simulink model "FullFMS_2026_02_25_V0_4_8"  (R2026a)
settings: Solver=FixedStepAuto  StopTime=inf  FixedStep=0.01  MaxStep=0.01  RelTol=1e-2
PreLoadFcn:
  | load("BUS_CONFIG.mat")
libraries: opcualib x8
(part 3 of 5)

== stateflow chart FullFMS_2026_02_25_V0_4_8/Chart ==
  state Variable_Declaration
    state VarDeclaration_20
      entry:
      %Actuators
      Actuators_20.F_22_Led_On;
      Actuators_20.F_22_Led_Off;
      Actuators_20.F_22_Conveyor;
      Actuators_20.F_24_Release_FB;
      Actuators_20.F_25_Release_FB;
      Actuators_20.F_26_Release_FB;
      Actuators_20.F_27_Release_FB;
      Actuators_20.F_28_Release_FB;
      Actuators_20.F_29_Release_FB;
      %Control
      Control_20.C_24_CartDel;
      Control_20.C_24_CRoute_Out;
      Control_20.C_24_Request;
      Control_20.C_24_CRoute_In;
      Control_20.C_25_CartDel;
      Control_20.C_25_CRoute_Out;
      Control_20.C_25_Request;
      Control_20.C_25_CRoute_In;
      Control_20.C_26_CartDel;
      Control_20.C_26_CRoute_Out;
      Control_20.C_26_Request;
      Control_20.C_26_CRoute_In;
      Control_20.C_27_CartDel;
      Control_20.C_27_CRoute_Out;
      Control_20.C_27_Request;
      Control_20.C_27_CRoute_In;
      Control_20.C_28_CartDel;
      Control_20.C_28_CRoute_Out;
      Control_20.C_28_Request;
      Control_20.C_28_CRoute_In;
      Control_20.C_29_CartDel;
      Control_20.C_29_CRoute_Out;
      Control_20.C_29_Request;
      Control_20.C_29_CRoute_In;
      %Sensors
      Sensors_20.O_20_On;
      Sensors_20.O_20_Off;
      Sensors_20.O_20_Controler_On;
      Sensors_20.O_24_Cart_Stat;
      Sensors_20.O_24_Cart_Next;
      Sensors_20.O_24_Optic;
      Sensors_20.O_24_Count;
      Sensors_20.O_24_Pist_Bck;
      Sensors_20.O_25_Cart_Stat;
      Sensors_20.O_25_Cart_Next;
      Sensors_20.O_25_Optic;
      Sensors_20.O_25_Count;
      Sensors_20.O_25_Pist_Bck;
      Sensors_20.O_26_Cart_Stat;
      Sensors_20.O_26_Cart_Next;
      Sensors_20.O_26_Optic;
      Sensors_20.O_26_Count;
      Sensors_20.O_26_Pist_Bck;
      Sensors_20.O_27_Cart_Stat;
      Sensors_20.O_27_Cart_Next;
      Sensors_20.O_27_Optic;
      Sensors_20.O_27_Count;
      Sensors_20.O_27_Pist_Bck;
      Sensors_20.O_28_Cart_Stat;
      Sensors_20.O_28_Cart_Next;
      Sensors_20.O_28_Optic;
      Sensors_20.O_28_Count;
      Sensors_20.O_28_Pist_Bck;
      Sensors_20.O_29_Cart_Stat;
      Sensors_20.O_29_Cart_Next;
      Sensors_20.O_29_Optic;
      Sensors_20.O_29_Count;
      Sensors_20.O_29_Pist_Bck;
    state VarDeclaration_30
      entry:
      %Actuators
      Actuators_30.F_33_Led_Start;
      Actuators_30.F_33_Led_Reset;
      Actuators_30.F_33_Led_Extra1;
      Actuators_30.F_33_Led_Extra2;
      Actuators_30.F_33_Spring_Cyl;
      Actuators_30.F_33_Cover_Cyl;
      %AS-i
      AS_i_30.A_34_Request;
      AS_i_30.A_34_No_Cart;
      AS_i_30.A_34_Cart_Full;
      AS_i_30.A_34_CRoute_Out;
      AS_i_30.A_32_RoboCartID;
      AS_i_30.A_34_Cart_Stat;
      AS_i_30.A_34_Cart_Next;
      AS_i_30.A_34_Optic;
      AS_i_30.A_34_Count;
      AS_i_30.A_34_Pist_Bck;
      AS_i_30.A_34_Release_FB;
      AS_i_30.A_34_CRoute_In;
      %Control
      Control_30.C_30_Robot1;
      Control_30.C_30_Robot2;
      Control_30.C_35_Part_Del;
      %Sensors
      Sensors_30.O_31_Start;
      Sensors_30.O_31_Stop;
      Sensors_30.O_31_Reset;
      Sensors_30.O_31_Part_in_Claw;
      Sensors_30.O_31_Orientation;
      Sensors_30.O_32_Sp_Cyl_Bck;
      Sensors_30.O_32_Sp_Cyl_Fwd;
      Sensors_30.O_32_Co_Cyl_Bck;
      Sensors_30.O_32_Co_Cyl_Fwd;
      Sensors_30.O_32_Sp_PickUp;
      Sensors_30.O_32_Co_PickUp;
      Sensors_30.O_32_CoMag_Empty;
    state VarDeclaration_40
      entry:
      %Actuators
      Actuators_40.F_43_Led_Start;
      Actuators_40.F_43_Led_Reset;
      Actuators_40.F_43_Led_Extra1;
      Actuators_40.F_43_Led_Extra2;
      Actuators_40.F_43_Panel_O4;
      Actuators_40.F_43_Panel_O5;
      Actuators_40.F_43_Panel_O6;
      Actuators_40.F_43_Panel_O7;
      %AS-i
      AS_i_40.A_44_Request;
      AS_i_40.A_44_No_Cart;
      AS_i_40.A_44_Cart_Full;
      AS_i_40.A_44_CRoute_Out;
      AS_i_40.A_43_StorCartID;
      AS_i_40.A_44_Cart_Stat;
      AS_i_40.A_44_Cart_Next;
      AS_i_40.A_44_Optic;
      AS_i_40.A_44_Count;
      AS_i_40.A_44_Pist_Bck;
      AS_i_40.A_44_Release_FB;
      AS_i_40.A_44_CRoute_In;
      %Control
      Control_40.C_45_Initialization;
      Control_40.C_42_Profibus;
      Control_40.C_45_Start;
      Control_40.C_45_StorePart;
      Control_40.C_45_RetrievePart;
      %Sensors
      Sensors_40.O_41_Start;
      Sensors_40.O_41_Stop;
      Sensors_40.O_41_Key_Pos;
      Sensors_40.O_41_Reset;
      Sensors_40.O_41_Panel_I4;
      Sensors_40.O_41_Panel_I5;
      Sensors_40.O_41_Panel_I6;
      Sensors_40.O_41_Panel_I7;
    state VarDeclaration_50
      entry:
      %Actuators
      Actuators_50.F_52_Claw_2_Del;
      Actuators_50.F_52_Claw_2_Cart;
      Actuators_50.F_52_Claw_Down;
      Actuators_50.F_52_Close_Claw;
      Actuators_50.F_53_Led_Start;
      Actuators_50.F_53_Led_Reset;
      Actuators_50.F_53_Led_Extra1;
      Actuators_50.F_53_Led_Extra2;
      Actuators_50.F_53_Panel_O4;
      Actuators_50.F_53_Panel_O5;
      Actuators_50.F_53_Panel_O6;
      Actuators_50.F_53_Panel_O7;
      %AS-i
      AS_i_50.A_54_Request;
      AS_i_50.A_54_No_Cart;
      AS_i_50.A_54_Cart_Full;
      AS_i_50.A_54_CRoute_Out;
      AS_i_50.A_53_SortCartID;
      AS_i_50.A_54_Cart_Stat;
      AS_i_50.A_54_Cart_Next;
      AS_i_50.A_54_Optic;
      AS_i_50.A_54_Count;
      AS_i_50.A_54_Pist_Bck;
      AS_i_50.A_54_Release_FB;
      AS_i_50.A_54_CRoute_In;
      %Control
      Control_50.C_55_Initialization;
      Control_50.C_55_PD_Sort;
      Control_50.C_52_Profibus;
      Control_50.C_55_Start;
      Control_50.C_55_Cart2Del;
      %Sensors
      Sensors_50.O_50_Part_Reserve;
      Sensors_50.O_50_Claw_Cart;
      Sensors_50.O_50_Claw_Del;
      Sensors_50.O_50_Claw_Reserve;
      Sensors_50.O_50_Claw_Low;
      Sensors_50.O_50_Claw_High;
      Sensors_50.O_50_Part_in_Claw;
      Sensors_50.O_51_Start;
      Sensors_50.O_51_Stop;
      Sensors_50.O_51_Key_Pos;
      Sensors_50.O_51_Reset;
      Sensors_50.O_51_Panel_I4;
      Sensors_50.O_51_Panel_I5;
      Sensors_50.O_51_Panel_I6;
      Sensors_50.O_51_Panel_I7;
    state VarDeclaration_60
      entry:
      %Actuators
      Actuators_60.F_62_Conveyor;
      Actuators_60.F_62_P1;
      Actuators_60.F_62_P2;
      Actuators_60.F_62_Identify;
      Actuators_60.F_63_Led_Start;
      Actuators_60.F_63_Led_Reset;
      Actuators_60.F_63_Led_Extra1;
      Actuators_60.F_63_Led_Extra2;
      Actuators_60.F_63_Panel_O4;
      Actuators_60.F_63_Panel_O5;
      Actuators_60.F_63_Panel_O6;
      Actuators_60.F_63_Panel_O7;
      %Control
      Control_60.C_65_Initialization;
      Control_60.C_65_ID_1;
      Control_60.C_65_ID_2;
      Control_60.C_65_Part_Sorted;
      Control_60.C_62_Profibus;
      Control_60.C_65_RBS_Output;
      Control_60.C_65_RSB_Output;
      Control_60.C_65_BRS_Output;
      Control_60.C_65_BSR_Output;
      Control_60.C_65_SRB_Output;
      Control_60.C_65_SBR_Output;
      %Sensors
      Sensors_60.O_60_SPart;
      Sensors_60.O_60_SInd;
      Sensors_60.O_60_SPhoto;
      Sensors_60.O_60_Part_Pass;
      Sensors_60.O_60_SL1_Bck;
      Sensors_60.O_60_SL1_Fwd;
      Sensors_60.O_60_SL2_Bck;
      Sensors_60.O_60_SL2_Fwd;
      Sensors_60.O_61_Start;
      Sensors_60.O_61_Stop;
      Sensors_60.O_61_Key_Pos;
      Sensors_60.O_61_Reset;
      Sensors_60.O_61_Panel_I4;
      Sensors_60.O_61_Panel_I5;
      Sensors_60.O_61_Panel_I6;
      Sensors_60.O_61_Panel_I7;
    state VarDeclaration_70
      entry:
      %Actuators
      Actuators_70.F_72_Elev_Down;
      Actuators_70.F_72_Elev_Up;
      Actuators_70.F_72_Eject_Part;
      Actuators_70.F_72_Air_On;
      Actuators_70.F_73_Led_Start;
      Actuators_70.F_73_Led_Reset;
      Actuators_70.F_73_Led_Extra1;
      Actuators_70.F_73_Led_Extra2;
      Actuators_70.F_73_Panel_O4;
      Actuators_70.F_73_Panel_O5;
      Actuators_70.F_73_Panel_O6;
      Actuators_70.F_73_Panel_O7;
      %AS-i
      AS_i_70.A_74_Request;
      AS_i_70.A_74_No_Cart;
      AS_i_70.A_74_Cart_Full;
      AS_i_70.A_74_CRoute_Out;
      AS_i_70.A_74_CRoute_In80;
      AS_i_70.A_73_TestCartID;
      AS_i_70.A_74_Cart_Stat;
      AS_i_70.A_74_Cart_Next;
      AS_i_70.A_74_Optic;
      AS_i_70.A_74_Count;
      AS_i_70.A_74_Pist_Bck;
      AS_i_70.A_74_Release_FB;
      AS_i_70.A_74_CRoute_In;
      %Control
      Control_70.C_75_Initialization;
      Control_70.C_75_ID_Delivery1;
      Control_70.C_75_ID_Delivery2;
      Control_70.C_75_Part_Del;
      Control_70.C_75_RQ_Part_Del;
      Control_70.C_75_RQ_Wrong;
      Control_70.C_75_Identified80;
      Control_70.C_75_Requested80;
      Control_70.C_72_Profibus;
      Control_70.C_75_RQ_Delivery1;
      Control_70.C_75_RQ_Delivery2;
      Control_70.C_75_Identified;
      Control_70.C_75_Requested;
      %Sensors
      Sensors_70.O_70_SInductive;
      Sensors_70.O_70_SPart;
      Sensors_70.O_70_SStation;
      Sensors_70.O_70_SPart_Height;
      Sensors_70.O_70_Elev_High;
      Sensors_70.O_70_Elev_Low;
      Sensors_70.O_70_Pist_Bck;
      Sensors_70.O_71_Start;
      Sensors_70.O_71_Stop;
      Sensors_70.O_71_Key_Pos;
      Sensors_70.O_71_Reset;
      Sensors_70.O_71_Panel_I4;
      Sensors_70.O_71_Panel_I5;
      Sensors_70.O_71_Panel_I6;
      Sensors_70.O_71_Panel_I7;
    state VarDeclaration_80
      entry:
      %Actuators
      Actuators_80.F_82_Pist_Adv;
      Actuators_80.F_82_Suction_On;
      Actuators_80.F_82_Suction_Off;
      Actuators_80.F_82_Arm_2_Del;
      Actuators_80.F_82_Arm_2_Mag;
      Actuators_80.F_83_Led_Start;
      Actuators_80.F_83_Led_Reset;
      Actuators_80.F_83_Led_Extra1;
      Actuators_80.F_83_Led_Extra2;
      Actuators_80.F_83_Panel_O4;
      Actuators_80.F_83_Panel_O5;
      Actuators_80.F_83_Panel_O6;
      Actuators_80.F_83_Panel_O7;
      %Control
      Control_80.C_85_Initialization;
      Control_80.C_85_Part_Del;
      Control_80.C_85_Part_Mag;
      Control_80.C_86_Mag_Parts;
      Control_80.C_87_RQ_MParts;
      Control_80.C_82_Profibus;
      Control_80.C_83_RQ_Parts;
      Control_80.C_85_Start;
      Control_80.C_85_Single;
      Control_80.C_85_Continuous;
      Control_80.C_85_Counted;
      %Sensors
      Sensors_80.O_80_Mag_Full;
      Sensors_80.O_80_Pist_Bck;
      Sensors_80.O_80_Pist_Fwd;
      Sensors_80.O_80_Part_Stuck;
      Sensors_80.O_80_Arm_Mag;
      Sensors_80.O_80_Arm_Del;
      Sensors_80.O_80_Mag_Empty;
      Sensors_80.O_81_Start;
      Sensors_80.O_81_Stop;,
      Sensors_80.O_81_Key_Pos;
      Sensors_80.O_81_Reset;
      Sensors_80.O_81_Panel_I4;
      Sensors_80.O_81_Panel_I5;
      Sensors_80.O_81_Panel_I6;
      Sensors_80.O_81_Panel_I7;
    state VarDeclaration_90
      entry:
      %Actuators
      Actuators_90.F_92_Claw_2_Cart;
      Actuators_90.F_92_Claw_2_Del;
      Actuators_90.F_92_Claw_Down;
      Actuators_90.F_92_Close_Claw;
      Actuators_90.F_93_Led_Start;
      Actuators_90.F_93_Led_Reset;
      Actuators_90.F_93_Led_Extra1;
      Actuators_90.F_93_Led_Extra2;
      Actuators_90.F_93_Panel_O4;
      Actuators_90.F_93_Panel_O5;
      Actuators_90.F_93_Panel_O6;
      Actuators_90.F_93_Panel_O7;
      %AS-i
      AS_i_90.A_94_Request;
      AS_i_90.A_94_No_Cart;
      AS_i_90.A_94_Cart_Full;
      AS_i_90.A_94_CRoute_Out;
      AS_i_90.A_93_ProcCartID;
      AS_i_90.A_94_Cart_Stat;
      AS_i_90.A_94_Cart_Next;
      AS_i_90.A_94_Optic;
      AS_i_90.A_94_Count;
      AS_i_90.A_94_Pist_Bck;
      AS_i_90.A_94_Release_FB;
      AS_i_90.A_94_CRoute_In;
      %Control
      Control_90.C_95_Initialization;
      Control_90.C_95_PD_Proc;
      Control_90.C_95_PD_Cart;
      Control_90.C_92_Profibus;
      Control_90.C_95_Start;
      Control_90.C_95_Cart2Del;
      Control_90.C_95_Del2Cart;
      %Sensors
      Sensors_90.O_90_Part_Reserve;
      Sensors_90.O_90_Claw_Del;
      Sensors_90.O_90_Claw_Cart;
      Sensors_90.O_90_Claw_Reserve;
      Sensors_90.O_90_Claw_Low;
      Sensors_90.O_90_Claw_High;
      Sensors_90.O_90_Part_in_Claw;
      Sensors_90.O_91_Start;
      Sensors_90.O_91_Stop;
      Sensors_90.O_91_Key_Pos;
      Sensors_90.O_91_Reset;
      Sensors_90.O_91_Panel_I4;
      Sensors_90.O_91_Panel_I5;
      Sensors_90.O_91_Panel_I6;
      Sensors_90.O_91_Panel_I7;
    state VarDeclaration_100
      entry:
      %Actuators
      Actuators_100.F_102_Drill_On;
      Actuators_100.F_102_RT_On;
      Actuators_100.F_102_Drill_Down;
      Actuators_100.F_102_Drill_Up;
      Actuators_100.F_102_Drill_Pin;
      Actuators_100.F_102_Test_Pin;
      Actuators_100.F_103_Led_Start;
      Actuators_100.F_103_Led_Reset;
      Actuators_100.F_103_Led_Extra1;
      Actuators_100.F_103_Led_Extra2;
      Actuators_100.F_103_Panel_O4;
      Actuators_100.F_103_Panel_O5;
      Actuators_100.F_103_Panel_O6;
      Actuators_100.F_103_Panel_O7;
      %Control
      Control_100.C_105_Initialization;
      Control_100.C_105_Part_ready;
      Control_100.C_105_Test_Ok;
      Control_100.C_105_Test_Fail;
      Control_100.C_106_RT_Counter;
      Control_100.C_102_Profibus;
      Control_100.C_103_RQ_Turns;
      Control_100.C_105_Start;
      Control_100.C_105_Test;
      Control_100.C_105_TestDrill;
      Control_100.C_105_Rotation;
      %Sensors
      Sensors_100.O_100_PInit_Pos;
      Sensors_100.O_100_PDrill_Pos;
      Sensors_100.O_100_PTest_Pos;
      Sensors_100.O_100_SDrill_High;
      Sensors_100.O_100_SDrill_Low;
      Sensors_100.O_100_RT_Sensor;
      Sensors_100.O_100_PTest_Ok;
      Sensors_100.O_101_Start;
      Sensors_100.O_101_Stop;
      Sensors_100.O_101_Key_Pos;
      Sensors_100.O_101_Reset;
      Sensors_100.O_101_Panel_I4;
      Sensors_100.O_101_Panel_I5;
      Sensors_100.O_101_Panel_I6;
      Sensors_100.O_101_Panel_I7;
    (default) -> VarDeclaration_20
    VarDeclaration_60 -> VarDeclaration_70
    VarDeclaration_30 -> VarDeclaration_40
    VarDeclaration_40 -> VarDeclaration_50
    VarDeclaration_70 -> VarDeclaration_80
    VarDeclaration_80 -> VarDeclaration_90
    VarDeclaration_50 -> VarDeclaration_60
    VarDeclaration_90 -> VarDeclaration_100
    VarDeclaration_20 -> VarDeclaration_30
  note: Sorting [60]
  state BRS Output
    state STATE1
      entry:
      StatusBRS_1 = false;
      during:
      % Configuracao da estacao: so este bloco fica ativo se o bit dele estiver ligado
      if Control_60.C_65_Initialization && Control_60.C_65_BRS_Output
      StatusBRS_1 = true;
      else
      StatusBRS_1 = false;
      end
    state ESTATE2
      entry:
      StatusBRS_2 = false;
      during:
      % Janela de identificacao da peca (T1 = 2s no ladder)
      if Control_50.C_55_PD_Sort
      StatusBRS_2 = true;
      else
      StatusBRS_2 = false;
      end
    state ESTATE3
      entry:
      StatusBRS_3 = false;
      during:
      % Preta: SL1 avanca | Vermelha: SL2 avanca | Prata: ambas recuadas
      if ((Control_60.C_65_ID_1 && ~Control_60.C_65_ID_2) && Sensors_60.O_60_SL1_Fwd) || ...
      ((Control_60.C_65_ID_1 && Control_60.C_65_ID_2) && Sensors_60.O_60_SL2_Fwd) || ...
      ((~Control_60.C_65_ID_1 && Control_60.C_65_ID_2) && Sensors_60.O_60_SL1_Bck && Sensors_60.O_60_SL2_Bck)
      StatusBRS_3 = true;
      else
      StatusBRS_3 = false;
      end
    state ESTATE4
      entry:
      StatusBRS_4 = false;
      during:
      % Pino de identificacao acionado (LEITURA do CLP - sombra nao comanda)
      if Actuators_60.F_62_Identify
      StatusBRS_4 = true;
      else
      StatusBRS_4 = false;
      end
    state ESTATE5
      entry:
      StatusBRS_5 = false;
      during:
      % Pino recuado: ciclo concluido, pronto para a proxima peca
      if ~Actuators_60.F_62_Identify
      StatusBRS_5 = true;
      else
      StatusBRS_5 = false;
      end
    (default) -> BRS.STATE1
    BRS.ESTATE2 -> BRS.ESTATE3 : [(Control_60.C_65_ID_1 == true || Control_60.C_65_ID_2 == true || after(2, sec)) && StatusBRS_2 == true]
    BRS.ESTATE5 -> BRS.STATE1 : [StatusBRS_5 == true]
    BRS.ESTATE3 -> BRS.ESTATE4 : [StatusBRS_3 == true]
    BRS.STATE1 -> BRS.ESTATE2 : [Control_50.C_55_PD_Sort == true && Sensors_50.O_50_Claw_Del == true && StatusBRS_1 == true]
    BRS.ESTATE4 -> BRS.ESTATE5 : [Sensors_60.O_60_Part_Pass == true && StatusBRS_4 == true]
  state Start
    during:
    Control_20.C_24_Request
  note: Conveyor
  state CartToTesting
    state StartsProcess
      entry:
      Status1_2 = false;
      during:
      Actuators_20.F_22_Conveyor;
      AS_i_50.A_53_SortCartID;
      AS_i_50.A_54_Pist_Bck;
      AS_i_50.A_54_Release_FB;
      if Actuators_20.F_22_Conveyor && ...
      AS_i_50.A_53_SortCartID == 0 && ...
      AS_i_50.A_54_Pist_Bck && ...
      AS_i_50.A_54_Release_FB
      Status1_2 = true;
      else
      Status1_2 = false;
      end
    state CartStartsMoving
      entry:
      Status1_3 = false;
      during:
      Actuators_50.F_53_Led_Extra1;
      AS_i_50.A_54_No_Cart;
      AS_i_50.A_54_Cart_Stat;
      if Actuators_50.F_53_Led_Extra1 && ...
      AS_i_50.A_54_No_Cart && ...
      ~AS_i_50.A_54_Cart_Stat
      Status1_3 = true;
      else
      Status1_3 = false;
      end
    state CartGetsNearNextStation
      entry:
      Status1_4 = false;
      during:
      AS_i_50.A_54_Cart_Next;
      AS_i_50.A_54_Pist_Bck;
      AS_i_50.A_54_Release_FB;
      if AS_i_50.A_54_Cart_Next && ...
      ~AS_i_50.A_54_Pist_Bck & ...
      ~AS_i_50.A_54_Release_FB
      Status1_4 = true;
      else
      Status1_4 = false;
      end
    state DetectionofCartNumberinStation
      entry:
      Status1_5 = false;
      during:
      AS_i_70.A_73_TestCartID
      if AS_i_70.A_73_TestCartID ~= 0
      Status1_5 = true;
      else
      Status1_5 = false;
      end
    state CartPassesNextStation
      entry:
      Status1_6 = false;
      during:
      AS_i_50.A_54_Cart_Next;
      if ~AS_i_50.A_54_Cart_Next;
      Status1_6 = true;
      else
      Status1_6 = false;
      end
    state CartArrivesinNextStation
      entry:
      Status1_7 = false;
      during:
      Control_20.C_24_CartDel;
      Actuators_70.F_73_Led_Extra1;
      AS_i_70.A_74_No_Cart;
      AS_i_70.A_74_Cart_Stat;
      AS_i_70.A_74_CRoute_In;
      if Control_20.C_24_CartDel;
      ~Actuators_70.F_73_Led_Extra1;
      ~AS_i_70.A_74_No_Cart;
      AS_i_70.A_74_Cart_Stat;
      AS_i_70.A_74_CRoute_In;
      Status1_7 = true;
      else
      Status1_7 = false;
      end
    state InitialCondition
      entry:
      Status1_1 = false;
      during:
      Actuators_20.F_22_Conveyor;
      AS_i_50.A_53_SortCartID;
      AS_i_50.A_54_Pist_Bck;
      AS_i_50.A_54_Release_FB;
      if ~Actuators_20.F_22_Conveyor && ...
      ~AS_i_50.A_53_SortCartID ~= 0 && ...
      ~AS_i_50.A_54_Pist_Bck && ...
      ~AS_i_50.A_54_Release_FB
      Status1_1 = true;
      else
      Status1_1 = false;
      end
    state T1
      during:
      Control_20.C_24_Request
    state T3
      during:
      Control_20.C_24_CartDel
    state T2
      during:
      AS_i_70.A_74_CRoute_In
    CartToTesting.CartStartsMoving -> CartToTesting.CartGetsNearNextStation : [Sensors_20.O_29_Cart_Next == true && ...
        | Status1_3 == true]
    CartToTesting.CartPassesNextStation -> CartToTesting.CartArrivesinNextStation : [Sensors_20.O_24_Cart_Stat == true && ...
        | Status1_6 == true]
    (default) -> CartToTesting.InitialCondition
    CartToTesting.InitialCondition -> CartToTesting.StartsProcess : [Control_20.C_24_Request == true && ...
        |  Status1_1 == true]
    CartToTesting.CartGetsNearNextStation -> CartToTesting.DetectionofCartNumberinStation : [Sensors_20.O_29_Count == true && ...
        | Status1_4 == true]
    CartToTesting.DetectionofCartNumberinStation -> CartToTesting.CartPassesNextStation : [Sensors_20.O_29_Cart_Next == false && ...
        | Status1_5 == true]
    CartToTesting.StartsProcess -> CartToTesting.CartStartsMoving [order 1] : [Sensors_20.O_29_Cart_Stat == false && ...
        |  Status1_2 == true]
    CartToTesting.StartsProcess -> CartToTesting.T1 [order 2] : [after(2, sec)]
    CartToTesting.CartArrivesinNextStation -> (junction 582)
    (junction 582) -> CartToTesting.T3 [order 2] : [after(3,sec)]
    (junction 582) -> CartToTesting.T2 [order 1] : [after(2,sec)]
  note: Testing Station [70]
  note: Distribution Station [80]
  state Identified_Delivery
    state Part_HeightSensor
      entry:
      St_IdDl_3a_8 = false;
      during:
      Actuators_70.F_72_Eject_Part;
      Sensors_70.O_70_Pist_Bck;
      Sensors_70.O_70_SPart_Height
      if Actuators_70.F_72_Eject_Part && ...
      ~Sensors_70.O_70_Pist_Bck && ...
      ~Sensors_70.O_70_SPart_Height
      St_IdDl_3a_8 = true
      else
      St_IdDl_3a_8 = false
      end
    state Piston_Back
      entry:
      Status3a_10 = false;
      during:
      Actuators_70.F_72_Eject_Part
      if ~Actuators_70.F_72_Eject_Part
      Status3a_10 = true
      else
      Status3a_10 = false
      end
    state Elevator_StartsMovingDown
      entry:
      Status3a_11 = false;
      during:
      Actuators_70.F_72_Elev_Down;
      Actuators_70.F_72_Elev_Up;
      if Actuators_70.F_72_Elev_Down && ...
      ~Actuators_70.F_72_Elev_Up
      Status3a_11 = true
      else
      Status3a_11 = false
      end
    state Elevator_MiddleDown
      entry:
      Status3a_12 = false;
      during:
      Sensors_70.O_70_SStation;
      if ~Sensors_70.O_70_SStation
      Status3a_12 = true
      else
      Status3a_12 = false
      end
    state Elevator_InductiveDown
      entry:
      St_IdDl_3a_13 = false;
      during:
      Sensors_70.O_70_SInductive;
      if ~Sensors_70.O_70_SInductive
      St_IdDl_3a_13 = true
      else
      St_IdDl_3a_13 = false
      end
    state Pushes_Part
      entry:
      Status3a_7 = false;
      during:
      Actuators_70.F_72_Eject_Part;
      Actuators_70.F_72_Air_On;
      Sensors_70.O_70_SPart;
      if Actuators_70.F_72_Eject_Part && ...
      Actuators_70.F_72_Air_On && ...
      ~Sensors_70.O_70_SPart
      Status3a_7 = true
      else
      Status3a_7 = false
      end
    state InitialCondition
      entry:
      St_IdDl_3a_1 = false;
      during:
      AS_i_70.A_74_Cart_Full;
      Control_70.C_75_Initialization;
      Control_70.C_72_Profibus;
      Control_70.C_75_Identified;
      Sensors_70.O_70_SPart;
      Sensors_70.O_71_Key_Pos;
      if ~AS_i_70.A_74_Cart_Full && ...
      Control_70.C_75_Initialization && ...
      Control_70.C_72_Profibus && ...
      Control_70.C_75_Identified && ...
      ~Sensors_70.O_70_SPart && ...
      Sensors_70.O_71_Key_Pos
      St_IdDl_3a_1 = true;
      else
      St_IdDl_3a_1 = false;
      end
    state Part_Arrives
      entry:
      Status3a_2 = false;
      during:
      Control_70.C_75_ID_Delivery2;
      Sensors_70.O_70_SInductive;
      Sensors_70.O_70_SPart;
      Sensors_80.O_80_Arm_Mag;
      if Sensors_70.O_70_SPart && ...
      ((Sensors_70.O_70_SInductive && ...
      Control_70.C_75_ID_Delivery2) | ...
      (~Sensors_70.O_70_SInductive && ...
      ~Control_70.C_75_ID_Delivery2)) && ...
      ~Sensors_80.O_80_Arm_Mag
      Status3a_2 = true;
      else
      Status3a_2 =false;
      end
    state Elevator_Up
      entry:
      Status3a_3 = false;
      during:
      Actuators_70.F_72_Elev_Up;
      if Actuators_70.F_72_Elev_Up
      Status3a_3 = true
      else
      Status3a_3 = false
      end
    state Elevator_StartsMovingUp
      entry:
      Status3a_4 = false;
      during:
      Sensors_70.O_70_SInductive;
      if ~Sensors_70.O_70_SInductive
      Status3a_4 = true
      else
      Status3a_4 = false
      end
    state Elevator_MiddleUp
      entry:
      Status3a_5 = false;
      during:
      Sensors_70.O_70_SStation;
      if ~Sensors_70.O_70_SStation
      Status3a_5 = true
      else
      Status3a_5 = false
      end
    state Elevator_High_Identify_Part
      entry:
      Status3a_6 = false;
      during:
      MetalicPart;
      Control_70.C_75_ID_Delivery1;
      Control_70.C_75_ID_Delivery2;
      Sensors_70.O_70_SPart_Height;
      if MetalicPart && ...
      Control_70.C_75_ID_Delivery2 && ...
      ~Control_70.C_75_ID_Delivery1;
      Status3a_6 = true
      end
      if ~MetalicPart && ...
      Control_70.C_75_ID_Delivery1 && ...
      ((Sensors_70.O_70_SPart_Height && ...
      Control_70.C_75_ID_Delivery2) | ...
      (~Sensors_70.O_70_SPart_Height && ...
      ~Control_70.C_75_ID_Delivery2))
      Status3a_6=true
      end
    state Elevator_Down
      entry:
      Status3a_14 = false;
      during:
      AS_i_70.A_74_CRoute_Out;
      Actuators_70.F_72_Elev_Down;
      Control_70.C_75_Part_Del;
      if AS_i_70.A_74_CRoute_Out && ...
      ~Actuators_70.F_72_Elev_Down&& ...
      Control_70.C_75_Part_Del
      Status3a_14 = true
      else
      Status3a_14 = false
      end
    state Part_ArrivesAtCart
      entry:
      Status3a_9 = false;
      during:
      AS_i_70.A_74_Cart_Full;
      AS_i_70.A_74_Optic;
      Actuators_70.F_72_Air_On;
      Actuators_70.F_73_Led_Extra2
      if AS_i_70.A_74_Optic && ...
      AS_i_70.A_74_Cart_Full && ...
      ~Actuators_70.F_72_Air_On && ...
      Actuators_70.F_73_Led_Extra2;
      Status3a_9 = true
      else
      Status3a_9 = false
      end
    state End_Process
      entry:
      Status3a_15 = false;
      during:
      AS_i_70.A_74_CRoute_Out;
      if  ~AS_i_70.A_74_CRoute_Out;
      Status3a_15 = true
      else
      Status3a_15 = false
      end
    state Metalic_Identify
      entry:
      MetalicPart = false;
      during:
      Sensors_70.O_70_SInductive;
      if Sensors_70.O_70_SInductive
      MetalicPart = true
      else
      MetalicPart = false
      end
    (default) -> Identified_Delivery.InitialCondition
    Identified_Delivery.Elevator_StartsMovingDown -> Identified_Delivery.Elevator_MiddleDown : [Status3a_11 == true && ...
        | Sensors_70.O_70_SStation == true]
    Identified_Delivery.Piston_Back -> Identified_Delivery.Elevator_StartsMovingDown : [Status3a_10 == true && ...
        | Sensors_70.O_70_Pist_Bck == true]
    Identified_Delivery.Elevator_MiddleDown -> Identified_Delivery.Elevator_InductiveDown : [Status3a_12 == true && ...
        | Sensors_70.O_70_SInductive == true]
    Identified_Delivery.Part_Arrives -> Identified_Delivery.Elevator_Up : [Status3a_2 == true && ...
        | Sensors_80.O_80_Arm_Mag == true ]
    Identified_Delivery.Elevator_High_Identify_Part -> Identified_Delivery.Pushes_Part : [Status3a_6 == true && ...
        | after (2,sec)]
    Identified_Delivery.Pushes_Part -> Identified_Delivery.Part_HeightSensor : [Status3a_7 == true && ...
        | Sensors_70.O_70_Pist_Bck == false]
    Identified_Delivery.Elevator_Up -> Identified_Delivery.Elevator_StartsMovingUp : [Status3a_3 == true && ...
        | Sensors_70.O_70_SInductive == true ]
    Identified_Delivery.Elevator_InductiveDown -> Identified_Delivery.Elevator_Down : [St_IdDl_3a_13 == true && ...
        | Sensors_70.O_70_Elev_Low == true]
    Identified_Delivery.Part_HeightSensor -> (junction 1354)
    (junction 1354) -> Identified_Delivery.Piston_Back [order 1] : [St_IdDl_3a_8 == true && ...
        | after (2,sec)]
    Identified_Delivery.Elevator_StartsMovingUp -> Identified_Delivery.Elevator_MiddleUp : [Status3a_4 == true && ...
        | Sensors_70.O_70_SStation == true]
    Identified_Delivery.Elevator_MiddleUp -> Identified_Delivery.Elevator_High_Identify_Part : [Status3a_5 == true && ...
        | Sensors_70.O_70_Elev_High == true]
    Identified_Delivery.InitialCondition -> (junction 1348) : [St_IdDl_3a_1 == true && ...
        | Sensors_70.O_70_SPart == true]
    (junction 1348) -> Identified_Delivery.Part_Arrives [order 1]
    (junction 1354) -> (junction 1356) [order 2] : [St_IdDl_3a_8 == true && ...
        | AS_i_70.A_74_Optic == true]
    (junction 1348) -> (junction 1350) [order 2]
    Identified_Delivery.Elevator_Down -> Identified_Delivery.End_Process : after (2,sec)
    (junction 1356) -> Identified_Delivery.Part_ArrivesAtCart
    (junction 1350) -> Identified_Delivery.Metalic_Identify
  state Distribution_Single
    state PistonStartsMoveBackward
      entry:
      St_DSg0_2a_7 = false;
      during:
      Sensors_80.O_80_Pist_Fwd;
      if ~Sensors_80.O_80_Pist_Fwd
      St_DSg0_2a_7 = true;
      else
      St_DSg0_2a_7 = false;
      end
    state PartFed
      entry:
      St_DSg0_2a_6 = false;
      during:
      Actuators_80.F_82_Pist_Adv;
      if ~Actuators_80.F_82_Pist_Adv
      St_DSg0_2a_6 = true;
      else
      St_DSg0_2a_6 = false;
      end
    state ArmToMagazine
      entry:
      St_DSg0_2a_8 = false;
      during:
      Actuators_80.F_82_Arm_2_Mag;
      if Actuators_80.F_82_Arm_2_Mag
      St_DSg0_2a_8 = true;
      else
      St_DSg0_2a_8 = false;
      end
    state ArmCloseDeliver1
      entry:
      St_DSg0_2a_9 = false;
      during:
      Sensors_70.O_70_SStation;
      if Sensors_70.O_70_SStation
      St_DSg0_2a_9 = true;
      else
      St_DSg0_2a_9 = false;
      end
    state ArmArrives_PicksPart
      entry:
      St_DSg0_2a_10 = false;
      during:
      Actuators_80.F_82_Suction_On;
      Actuators_80.F_82_Arm_2_Mag;
      if Actuators_80.F_82_Suction_On && ...
      ~Actuators_80.F_82_Arm_2_Mag
      St_DSg0_2a_10 = true;
      else
      St_DSg0_2a_10 = false;
      end
    state ArmToDelivery1
      entry:
      St_DSg0_2a_11 = false;
      during:
      Actuators_80.F_82_Arm_2_Del
      if Actuators_80.F_82_Arm_2_Del
      St_DSg0_2a_11 = true;
      else
      St_DSg0_2a_11 = false;
      end
    state ArmCloseDelivery2
      entry:
      St_DSg0_2a_12 = false;
      during:
      Sensors_70.O_70_SStation;
      if Sensors_70.O_70_SStation
      St_DSg0_2a_12 = true;
      else
      St_DSg0_2a_12 = false;
      end
    state ArmArrives_DeliversPart
      entry:
      St_DSg0_2a_13 = false;
      during:
      Actuators_80.F_82_Suction_On;
      Actuators_80.F_82_Suction_Off;
      Actuators_80.F_82_Arm_2_Del;
      if ~Actuators_80.F_82_Suction_On && ...
      Actuators_80.F_82_Suction_Off && ...
      ~Actuators_80.F_82_Arm_2_Del
      St_DSg0_2a_13 = true;
      else
      St_DSg0_2a_13 = false;
      end
    state ArmToMagazine1
      entry:
      St_DSg0_2a_14 = false;
      during:
      Actuators_80.F_82_Suction_Off;
      Actuators_80.F_82_Arm_2_Mag;
      Actuators_80.F_83_Led_Extra1;
      Control_80.C_85_Part_Del;
      if ~Actuators_80.F_82_Suction_Off && ...
      Actuators_80.F_82_Arm_2_Mag && ...
      Actuators_80.F_83_Led_Extra1 && ...
      Control_80.C_85_Part_Del
      St_DSg0_2a_14 = true;
      else
      St_DSg0_2a_14 = false;
      end
    state ArmCloseDeliver3
      entry:
      St_DSg0_2a_15 = false;
      during:
      Sensors_70.O_70_SStation;
      if Sensors_70.O_70_SStation
      St_DSg0_2a_15 = true;
      else
      St_DSg0_2a_15 = false;
      end
    state ArmArrives_Finish
      entry:
      St_DSg0_2a_16 = false;
      during:
      Actuators_80.F_82_Arm_2_Mag;
      if ~Actuators_80.F_82_Arm_2_Mag;
      St_DSg0_2a_16 = true;
      else
      St_DSg0_2a_16 = false;
      end
    state InitialCondition
      entry:
      St_DSg0_2a_1 = false;
      during:
      Control_80.C_85_Initialization;
      Control_80.C_86_Mag_Parts;
      Control_80.C_82_Profibus;
      Control_80.C_85_Single;
      Sensors_80.O_80_Arm_Mag;
      Sensors_80.O_81_Key_Pos;
      if Control_80.C_85_Initialization&& ...
      Control_80.C_86_Mag_Parts ~= 0 && ...
      Control_80.C_82_Profibus && ...
      Control_80.C_85_Single && ...
      Sensors_80.O_80_Arm_Mag && ...
      Sensors_80.O_81_Key_Pos
      St_DSg0_2a_1 = true;
      else
      St_DSg0_2a_1 = false;
      end
    state ArmToDelivery
      entry:
      St_DSg0_2a_2 = false;
      during:
      Actuators_80.F_82_Arm_2_Del;
      if Actuators_80.F_82_Arm_2_Del
      St_DSg0_2a_2 = true;
      else
      St_DSg0_2a_2 = false;
      end
    state ArmCloseDelivery
      entry:
      St_DSg0_2a_3 = false;
      during:
      Sensors_70.O_70_SStation;
      if Sensors_70.O_70_SStation
      St_DSg0_2a_3 = true;
      else
      St_DSg0_2a_3 = false;
      end
    state ArmArrives_FeedsPart
      entry:
      St_DSg0_2a_4 = false;
      during:
      Actuators_80.F_82_Pist_Adv;
      Actuators_80.F_82_Arm_2_Del;
      if Actuators_80.F_82_Pist_Adv && ...
      ~Actuators_80.F_82_Arm_2_Del
      St_DSg0_2a_4 = true;
      else
      St_DSg0_2a_4 = false;
      end
    state PistonStartsMoveForward
      entry:
      St_DSg0_2a_5 = false;
      during:
      Sensors_80.O_80_Pist_Bck;
      if ~Sensors_80.O_80_Pist_Bck
      St_DSg0_2a_5 = true;
      else
      St_DSg0_2a_5 = false;
      end
    state T1
      during:
      Control_80.C_85_Part_Del
      Actuators_80.F_83_Led_Extra1
    (default) -> Distribution_Single.InitialCondition
    Distribution_Single.ArmToMagazine1 -> (junction 650)
    (junction 650) -> Distribution_Single.ArmCloseDeliver3 [order 1] : [Sensors_80.O_80_Arm_Del == false &&...
        |  St_DSg0_2a_14 == true]
    Distribution_Single.ArmToDelivery -> Distribution_Single.ArmCloseDelivery : [Sensors_80.O_80_Arm_Mag == false &&...
        |  St_DSg0_2a_2 == true]
    Distribution_Single.ArmCloseDelivery -> Distribution_Single.ArmArrives_FeedsPart : [Sensors_80.O_80_Arm_Del == true && ...
        | St_DSg0_2a_3 == true]
    Distribution_Single.ArmArrives_DeliversPart -> Distribution_Single.ArmToMagazine1 : [Sensors_80.O_80_Part_Stuck == false && ...
        | St_DSg0_2a_13 == true]
    Distribution_Single.ArmCloseDelivery2 -> Distribution_Single.ArmArrives_DeliversPart : [Sensors_80.O_80_Arm_Del == true && ...
        | St_DSg0_2a_12 == true]
    Distribution_Single.ArmArrives_FeedsPart -> Distribution_Single.PistonStartsMoveForward : [St_DSg0_2a_4 == true]
    Distribution_Single.PistonStartsMoveBackward -> Distribution_Single.ArmToMagazine : [Sensors_80.O_80_Pist_Bck == true && ...
        | St_DSg0_2a_7 == true]
    Distribution_Single.ArmCloseDeliver1 -> Distribution_Single.ArmArrives_PicksPart : [Sensors_80.O_80_Arm_Mag == true && ...
        | St_DSg0_2a_9 == true]
    Distribution_Single.PartFed -> Distribution_Single.PistonStartsMoveBackward : [St_DSg0_2a_6 == true]
    Distribution_Single.ArmToMagazine -> Distribution_Single.ArmCloseDeliver1 : [Sensors_80.O_80_Arm_Del == false &&...
        | St_DSg0_2a_8 == true]
    Distribution_Single.InitialCondition -> Distribution_Single.ArmToDelivery : [Sensors_80.O_81_Start == true | ...
        | Control_80.C_85_Start == true | ...
        | Control_70.C_75_RQ_Wrong == true | ...
        | (AS_i_70.A_74_CRoute_In80 == true && Sensors_80.O_81_Key_Pos == true) ]
    Distribution_Single.ArmCloseDeliver3 -> Distribution_Single.ArmArrives_Finish : [Sensors_80.O_80_Arm_Mag == true && ...
        | St_DSg0_2a_15 == true]
    Distribution_Single.ArmToDelivery1 -> Distribution_Single.ArmCloseDelivery2 : [Sensors_80.O_80_Arm_Mag == false &&...
        | St_DSg0_2a_11 == true]
    Distribution_Single.PistonStartsMoveForward -> Distribution_Single.PartFed : [Sensors_80.O_80_Pist_Fwd == true && ...
        | St_DSg0_2a_5 == true]
    Distribution_Single.ArmArrives_PicksPart -> Distribution_Single.ArmToDelivery1 : [Sensors_80.O_80_Part_Stuck == true && ...
        | St_DSg0_2a_10 == true]
    (junction 650) -> (junction 1222) [order 2] : after(4,sec)
    (junction 1222) -> Distribution_Single.T1
  state BSR Output
    state STATE1
      entry:
      StatusBSR_1 = false;
      during:
      % Configuracao da estacao: so este bloco fica ativo se o bit dele estiver ligado
      if Control_60.C_65_Initialization && Control_60.C_65_BSR_Output
      StatusBSR_1 = true;
      else
      StatusBSR_1 = false;
      end
    state ESTATE2
      entry:
      StatusBSR_2 = false;
      during:
      % Janela de identificacao da peca (T1 = 2s no ladder)
      if Control_50.C_55_PD_Sort
      StatusBSR_2 = true;
      else
      StatusBSR_2 = false;
      end
    state ESTATE3
      entry:
      StatusBSR_3 = false;
      during:
      % Preta: SL1 avanca | Prata: SL2 avanca | Vermelha: ambas recuadas
      if ((Control_60.C_65_ID_1 && ~Control_60.C_65_ID_2) && Sensors_60.O_60_SL1_Fwd) || ...
      ((~Control_60.C_65_ID_1 && Control_60.C_65_ID_2) && Sensors_60.O_60_SL2_Fwd) || ...
      ((Control_60.C_65_ID_1 && Control_60.C_65_ID_2) && Sensors_60.O_60_SL1_Bck && Sensors_60.O_60_SL2_Bck)
      StatusBSR_3 = true;
      else
      StatusBSR_3 = false;
      end
    state ESTATE4
      entry:
      StatusBSR_4 = false;
      during:
      % Pino de identificacao acionado (LEITURA do CLP - sombra nao comanda)
      if Actuators_60.F_62_Identify
      StatusBSR_4 = true;
      else
      StatusBSR_4 = false;
      end
    state ESTATE5
      entry:
      StatusBSR_5 = false;
      during:
      % Pino recuado: ciclo concluido, pronto para a proxima peca
      if ~Actuators_60.F_62_Identify
      StatusBSR_5 = true;
      else
      StatusBSR_5 = false;
      end
    (default) -> BSR.STATE1
    BSR.ESTATE4 -> BSR.ESTATE5 : [Sensors_60.O_60_Part_Pass == true && StatusBSR_4 == true]
    BSR.ESTATE3 -> BSR.ESTATE4 : [StatusBSR_3 == true]
    BSR.ESTATE2 -> BSR.ESTATE3 : [(Control_60.C_65_ID_1 == true || Control_60.C_65_ID_2 == true || after(2, sec)) && StatusBSR_2 == true]
    BSR.STATE1 -> BSR.ESTATE2 : [Control_50.C_55_PD_Sort == true && Sensors_50.O_50_Claw_Del == true && StatusBSR_1 == true]
    BSR.ESTATE5 -> BSR.STATE1 : [StatusBSR_5 == true]
  note: Handling 1 [50]
  state Distribution_Continuous
    state InitialCondition
      entry:
      St_DCt0_2b_1 = false;
      during:
      Control_80.C_85_Initialization;
      Control_80.C_86_Mag_Parts;
      Control_80.C_82_Profibus;
      Control_80.C_85_Continuous;
      Sensors_80.O_80_Arm_Mag;
      Sensors_80.O_81_Key_Pos;
      if Control_80.C_85_Initialization&& ...
      Control_80.C_86_Mag_Parts ~= 0 && ...
      Control_80.C_82_Profibus && ...
      Control_80.C_85_Continuous && ...
      Sensors_80.O_80_Arm_Mag && ...
      Sensors_80.O_81_Key_Pos
      St_DCt0_2a_1 = true;
      else
      St_DCt0_2b_1 = false;
      end
    state ArmToDelivery
      entry:
      St_DCt0_2b_2 = false;
      during:
      Actuators_80.F_82_Arm_2_Del
      if Actuators_80.F_82_Arm_2_Del
      St_DCt0_2b_2 = true;
      else
      St_DCt0_2b_2 = false;
      end
    state ArmCloseDelivery
      entry:
      St_DCt0_2b_3 = false;
      during:
      Sensors_70.O_70_SStation;
      if Sensors_70.O_70_SStation
      St_DCt0_2b_3 = true;
      else
      St_DCt0_2b_3 = false;
      end
    state ArmArrives_FeedsPart
      entry:
      St_DCt0_2b_4 = false;
      during:
      Actuators_80.F_82_Pist_Adv;
      Actuators_80.F_82_Arm_2_Del;
      if Actuators_80.F_82_Pist_Adv && ...
      ~Actuators_80.F_82_Arm_2_Del
      St_DCt0_2b_4 = true;
      else
      St_DCt0_2b_4 = false;
      end
    state PistonStartsMoveForward
      entry:
      St_DCt0_2b_5 = false;
      during:
      Sensors_80.O_80_Pist_Bck;
      if ~Sensors_80.O_80_Pist_Bck
      St_DCt0_2b_5 = true;
      else
      St_DCt0_2b_5 = false;
      end
    state PartFed
      entry:
      St_DCt0_2b_6 = false;
      during:
      Actuators_80.F_82_Pist_Adv;
      if ~Actuators_80.F_82_Pist_Adv
      St_DCt0_2b_6 = true;
      else
      St_DCt0_2b_6 = false;
      end
    state PistonStartsMoveBackward
      entry:
      St_DCt0_2b_7 = false;
      during:
      Sensors_80.O_80_Pist_Fwd;
      if ~Sensors_80.O_80_Pist_Fwd
      St_DCt0_2b_7 = true;
      else
      St_DCt0_2b_7 = false;
      end
    state ArmToMagazine
      entry:
      St_DCt0_2b_8 = false;
      during:
      Actuators_80.F_82_Arm_2_Mag;
      if Actuators_80.F_82_Arm_2_Mag
      St_DCt0_2b_8 = true;
      else
      St_DCt0_2b_8 = false;
      end
    state ArmCloseDeliver1
      entry:
      St_DCt0_2b_9 = false;
      during:
      Sensors_70.O_70_SStation;
      if Sensors_70.O_70_SStation
      St_DCt0_2b_9 = true;
      else
      St_DCt0_2b_9 = false;
      end
    state ArmArrives_PicksPart
      entry:
      St_DCt0_2b_10 = false;
      during:
      Actuators_80.F_82_Suction_On;
      Actuators_80.F_82_Arm_2_Mag;
      if Actuators_80.F_82_Suction_On && ...
      ~Actuators_80.F_82_Arm_2_Mag
      St_DCt0_2b_10 = true;
      else
      St_DCt0_2b_10 = false;
      end
    state ArmToDelivery1
      entry:
      St_DCt0_2b_11 = false;
      during:
      Actuators_80.F_82_Arm_2_Del
      if Actuators_80.F_82_Arm_2_Del
      St_DCt0_2b_11 = true;
      else
      St_DCt0_2b_11 = false;
      end
    state ArmCloseDelivery2
      entry:
      St_DCt0_2b_12 = false;
      during:
      Sensors_70.O_70_SStation;
      if Sensors_70.O_70_SStation
      St_DCt0_2b_12 = true;
      else
      St_DCt0_2b_12 = false;
      end
    state ArmArrives_DeliversPart
      entry:
      St_DCt0_2b_13 = false;
      during:
      Actuators_80.F_82_Suction_On;
      Actuators_80.F_82_Suction_Off;
      Actuators_80.F_82_Arm_2_Del;
      if ~Actuators_80.F_82_Suction_On && ...
      Actuators_80.F_82_Suction_Off && ...
      ~Actuators_80.F_82_Arm_2_Del
      St_DCt0_2b_13 = true;
      else
      St_DCt0_2b_13 = false;
      end
    state PartDel_CheckLoop
      entry:
      LoopDistCont = false;
      during:
      Control_80.C_85_Part_Del
      Control_80.C_86_Mag_Parts
      if Control_80.C_85_Part_Del && ...
      Control_80.C_86_Mag_Parts ~= 0
      LoopDistCont = true;
      else
      LoopDistCont = false;
      end
    state ArmToMagazine1
      entry:
      St_DCt0_2b_14 = false;
      during:
      Actuators_80.F_82_Suction_Off;
      Actuators_80.F_82_Arm_2_Mag;
      Actuators_80.F_83_Led_Extra1;
      Control_80.C_85_Part_Del;
      if ~Actuators_80.F_82_Suction_Off && ...
      Actuators_80.F_82_Arm_2_Mag && ...
      Actuators_80.F_83_Led_Extra1 && ...
      Control_80.C_85_Part_Del
      St_DCt0_2b_14 = true;
      else
      St_DCt0_2b_14 = false;
      end
    state ArmCloseDeliver3
      entry:
      St_DCt0_2b_15 = false;
      during:
      Sensors_70.O_70_SStation;
      if Sensors_70.O_70_SStation
      St_DCt0_2b_15 = true;
      else
      St_DCt0_2b_15 = false;
      end
    state ArmArrives_Finish
      entry:
      St_DCt0_2b_16 = false;
      during:
      Actuators_80.F_82_Arm_2_Mag;
      if ~Actuators_80.F_82_Arm_2_Mag;
      St_DCt0_2b_16 = true;
      else
      St_DCt0_2b_16 = false;
      end
    state T1
      during:
      Control_80.C_85_Part_Del
      Actuators_80.F_83_Led_Extra1
    Distribution_Continuous.ArmArrives_PicksPart -> Distribution_Continuous.ArmToDelivery1 : [Sensors_80.O_80_Part_Stuck == true && ...
        | St_DCt0_2b_10 == true]
    Distribution_Continuous.ArmArrives_DeliversPart -> Distribution_Continuous.PartDel_CheckLoop : [Sensors_80.O_80_Part_Stuck == false && ...
        | St_DCt0_2b_13 == true]
    Distribution_Continuous.ArmCloseDelivery -> Distribution_Continuous.ArmArrives_FeedsPart : [Sensors_80.O_80_Arm_Del == true && ...
        | St_DCt0_2b_3 == true]
    Distribution_Continuous.ArmArrives_FeedsPart -> Distribution_Continuous.PistonStartsMoveForward : [St_DCt0_2b_4 == true]
    (default) -> Distribution_Continuous.InitialCondition
    Distribution_Continuous.PartFed -> Distribution_Continuous.PistonStartsMoveBackward : [St_DCt0_2b_6 == true]
    Distribution_Continuous.PistonStartsMoveForward -> Distribution_Continuous.PartFed : [Sensors_80.O_80_Pist_Fwd == true && ...
        | St_DCt0_2b_5 == true]
    Distribution_Continuous.ArmToDelivery -> Distribution_Continuous.ArmCloseDelivery : [Sensors_80.O_80_Arm_Mag == false &&...
        | St_DCt0_2a_2 == true]
    Distribution_Continuous.PistonStartsMoveBackward -> Distribution_Continuous.ArmToMagazine : [Sensors_80.O_80_Pist_Bck == true && ...
        | St_DCt0_2b_7 == true]
    Distribution_Continuous.ArmCloseDelivery2 -> Distribution_Continuous.ArmArrives_DeliversPart : [Sensors_80.O_80_Arm_Del == true && ...
        | St_DCt0_2b_12 == true]
    Distribution_Continuous.ArmToMagazine -> Distribution_Continuous.ArmCloseDeliver1 : [Sensors_80.O_80_Arm_Del == false &&...
        |  St_DCt0_2b_8 == true]
    Distribution_Continuous.ArmCloseDeliver1 -> Distribution_Continuous.ArmArrives_PicksPart : [Sensors_80.O_80_Arm_Mag == true && ...
        | St_DCt0_2b_9 == true]
    Distribution_Continuous.ArmToDelivery1 -> Distribution_Continuous.ArmCloseDelivery2 : [Sensors_80.O_80_Arm_Mag == false &&...
        |  St_DCt0_2b_11 == true]
    Distribution_Continuous.InitialCondition -> Distribution_Continuous.ArmToDelivery : [Sensors_80.O_81_Start == true | ...
        | Control_80.C_85_Start == true | ...
        | Control_70.C_75_RQ_Wrong == true | ...
        | (AS_i_70.A_74_CRoute_In80 == true && Sensors_80.O_81_Key_Pos == true) ]
    Distribution_Continuous.ArmToMagazine1 -> Distribution_Continuous.ArmCloseDeliver3 : [Sensors_80.O_80_Arm_Del == false &&...
        | St_DCt0_2b_14 == true]
    Distribution_Continuous.ArmCloseDeliver3 -> Distribution_Continuous.ArmArrives_Finish : [Sensors_80.O_80_Arm_Mag == true && ...
        | St_DCt0_2b_15 == true]
    Distribution_Continuous.PartDel_CheckLoop -> Distribution_Continuous.ArmToMagazine1 [order 2] : [LoopDistCont == false]
    (junction 708) -> Distribution_Continuous.ArmArrives_FeedsPart
    (junction 706) -> (junction 708)
    Distribution_Continuous.PartDel_CheckLoop -> (junction 707) [order 1] : [LoopDistCont == true]
    Distribution_Continuous.PartDel_CheckLoop -> Distribution_Continuous.T1 [order 3] : after(4,sec)
    (junction 707) -> (junction 706)
  state PartToProcessing2
    state FinishesProcess
      entry:
      St_P2P2_5_13 = false;
      during:
      Control_90.C_95_PD_Proc;
      if Control_90.C_95_PD_Proc
      St_P2P2_5_13 = true;
      else
      St_P2P2_5_13 = false;
      end
    state ClawBeginsAscend
      entry:
      St_P2P2_5_12 = false;
      during:
      Sensors_90.O_90_Part_in_Claw;
      if ~Sensors_90.O_90_Part_in_Claw
      St_P2P2_5_12 = true;
      else
      St_P2P2_5_12 = false;
      end
    state DeliversPart
      entry:
      St_P2P2_5_11 = false;
      during:
      Actuators_90.F_92_Claw_Down;
      Actuators_90.F_92_Close_Claw;
      if ~Actuators_90.F_92_Claw_Down && ...
      ~Actuators_90.F_92_Close_Claw
      St_P2P2_5_11 = true;
      else
      St_P2P2_5_11 = false;
      end
    state ClawDescent
      entry:
      St_P2P2_5_10 = false;
      during:
      Sensors_90.O_90_Claw_Low;
      Sensors_90.O_90_Claw_High;
      if Sensors_90.O_90_Claw_Low && ...
      ~Sensors_90.O_90_Claw_High
      St_P2P2_5_10 = true;
      else
      St_P2P2_5_10 = false;
      end
    state ArmArrives
      entry:
      St_P2P2_5_9 = false;
      during:
      Actuators_90.F_92_Claw_2_Del;
      Actuators_90.F_92_Claw_Down;
      if ~Actuators_90.F_92_Claw_2_Del && ...
      Actuators_90.F_92_Claw_Down
      St_P2P2_5_9 = true;
      else
      St_P2P2_5_9 = false;
      end
    state ArmPassesStorage
      entry:
      St_P2P2_5_8 = false;
      during:
      Sensors_90.O_90_Claw_Reserve;
      if ~Sensors_90.O_90_Claw_Reserve;
      St_P2P2_5_8 = true;
      else
      St_P2P2_5_8 = false;
      end
    state ArmStartsMovement
      entry:
      St_P2P2_5_7 = false;
      during:
      Sensors_90.O_90_Claw_Reserve;
      if Sensors_90.O_90_Claw_Reserve;
      St_P2P2_5_7 = true;
      else
      St_P2P2_5_7 = false;
      end
    state ClawFinishesAscend
      entry:
      St_P2P2_5_6 = false;
      during:
      Actuators_90.F_92_Claw_2_Del;
      if Actuators_90.F_92_Claw_2_Del
      St_P2P2_5_6 = true;
      else
      St_P2P2_5_6 = false;
      end
    state PartLeavesCart
      entry:
      St_P2P2_5_5 = false;
      during:
      AS_i_90.A_94_Cart_Full;
      if ~AS_i_90.A_94_Cart_Full
      St_P2P2_5_5 = true;
      else
      St_P2P2_5_5 = false;
      end
    state PartPickup_BeginsAscend
      entry:
      St_P2P2_5_4 = false;
      during:
      Actuators_90.F_92_Claw_Down;
      Sensors_90.O_90_Claw_Low;
      if ~Actuators_90.F_92_Claw_Down && ...
      ~Sensors_90.O_90_Claw_Low
      St_P2P2_5_4 = true;
      else
      St_P2P2_5_4 = false;
      end
    state ClawFinishesDescent
      entry:
      St_P2P2_5_3 = false;
      during:
      Actuators_90.F_92_Close_Claw;
      if Actuators_90.F_92_Close_Claw
      St_P2P2_5_3 = true;
      else
      St_P2P2_5_3 = false;
      end
    state ClawBeginsDescent
      entry:
      St_P2P2_5_2 = false;
      during:
      Actuators_90.F_92_Claw_Down;
      Control_90.C_95_PD_Proc;
      Control_90.C_95_PD_Cart;
      Sensors_90.O_90_Claw_High;
      if Actuators_90.F_92_Claw_Down && ...
      ~Control_90.C_95_PD_Proc && ...
      ~Control_90.C_95_PD_Cart && ...
      ~Sensors_90.O_90_Claw_High
      St_P2P2_5_2 = true;
      else
      St_P2P2_5_2 = false;
      end
    state InitialCondition
      entry:
      St_P2P2_5_1 = false;
      during:
      AS_i_90.A_94_Cart_Full;
      Control_90.C_95_Initialization;
      Control_90.C_95_Cart2Del;
      Control_90.C_92_Profibus;
      Sensors_90.O_91_Key_Pos;
      if AS_i_90.A_94_Cart_Full && ...
      Control_90.C_95_Initialization && ...
      Control_90.C_95_Cart2Del && ...
      Control_90.C_92_Profibus && ...
      Sensors_90.O_91_Key_Pos
      St_P2P2_5_1 = true;
      else
      St_P2P2_5_1 = false;
      end
    (default) -> PartToProcessing2.InitialCondition
    PartToProcessing2.ArmStartsMovement -> PartToProcessing2.ArmPassesStorage : [Sensors_90.O_90_Claw_Reserve == false && ...
        | St_P2P2_5_7 == true]
    PartToProcessing2.ClawBeginsAscend -> PartToProcessing2.FinishesProcess : [Sensors_90.O_90_Claw_High == true && ...
        | St_P2P2_5_12 == true]
    PartToProcessing2.DeliversPart -> PartToProcessing2.ClawBeginsAscend : [Sensors_90.O_90_Claw_Low && ...
        | St_P2P2_5_11 == true]
    PartToProcessing2.ArmArrives -> PartToProcessing2.ClawDescent : [Sensors_90.O_90_Claw_High == false && ...
        | St_P2P2_5_9 == true]
    PartToProcessing2.ClawFinishesAscend -> PartToProcessing2.ArmStartsMovement : [Sensors_90.O_90_Claw_Cart == false && ...
        | St_P2P2_5_6 == true]
    PartToProcessing2.ClawFinishesDescent -> PartToProcessing2.PartPickup_BeginsAscend : [Sensors_90.O_90_Part_in_Claw == true && ...
        | St_P2P2_5_3 == true]
    PartToProcessing2.PartLeavesCart -> PartToProcessing2.ClawFinishesAscend : [Sensors_90.O_90_Claw_High == true && ...
        | St_P2P2_5_5 == true]
    PartToProcessing2.PartPickup_BeginsAscend -> PartToProcessing2.PartLeavesCart : [AS_i_90.A_94_Optic == false && ...
        | St_P2P2_5_4 == true]
    PartToProcessing2.ClawDescent -> PartToProcessing2.DeliversPart : [Sensors_100.O_100_PInit_Pos == true && ...
        | St_P2P2_5_10 == true]
    PartToProcessing2.ClawBeginsDescent -> PartToProcessing2.ClawFinishesDescent : [Sensors_90.O_90_Claw_Low == true && ...
        | St_P2P2_5_2 == true]
    PartToProcessing2.InitialCondition -> PartToProcessing2.ClawBeginsDescent : [AS_i_90.A_94_CRoute_In == true && ...
        |  St_P2P2_5_1 == true]
    PartToProcessing2.ArmPassesStorage -> PartToProcessing2.ArmArrives : [Sensors_90.O_90_Claw_Del == true && ...
        | St_P2P2_5_8 == true]
  state Requested_Delivery
    state Part_HeightSensor
      entry:
      Status3b_8 = false;
      during:
      Actuators_70.F_72_Eject_Part;
      Sensors_70.O_70_Pist_Bck;
      Sensors_70.O_70_SPart_Height
      if Actuators_70.F_72_Eject_Part && ...
      ~Sensors_70.O_70_Pist_Bck && ...
      ~Sensors_70.O_70_SPart_Height
      Status3b_8 = true
      else
      Status3b_8 = false
      end
    state Piston_Back
      entry:
      Status3b_10 = false;
      during:
      Actuators_70.F_72_Eject_Part
      if ~Actuators_70.F_72_Eject_Part
      Status3b_10 = true
      else
      Status3b_10 = false
      end
    state Elevator_StartsMovingDown
      entry:
      Status3b_11 = false;
      during:
      Actuators_70.F_72_Elev_Down;
      Actuators_70.F_72_Elev_Up;
      if Actuators_70.F_72_Elev_Down && ...
      ~Actuators_70.F_72_Elev_Up
      Status3b_11 = true
      else
      Status3b_11 = false
      end
    state Elevator_MiddleDown
      entry:
      Status3b_12 = false;
      during:
      Sensors_70.O_70_SStation;
      if ~Sensors_70.O_70_SStation
      Status3b_12 = true
      else
      Status3b_12 = false
      end
    state Elevator_InductiveDown
      entry:
      Status3b_13 = false;
      during:
      Sensors_70.O_70_SInductive;
      if ~Sensors_70.O_70_SInductive
      Status3b_13 = true
      else
      Status3b_13 = false
      end
    state InitialCondition
      entry:
      Status3b_1 = false;
      during:
      AS_i_70.A_74_Cart_Full;
      Control_70.C_75_Initialization;
      Control_70.C_72_Profibus;
      Control_70.C_75_Requested;
      Sensors_70.O_70_SPart;
      Sensors_70.O_71_Key_Pos;
      if ~AS_i_70.A_74_Cart_Full && ...
      Control_70.C_75_Initialization && ...
      Control_70.C_72_Profibus && ...
      Control_70.C_75_Requested && ...
      ~Sensors_70.O_70_SPart && ...
      Sensors_70.O_71_Key_Pos
      Status3b_1 = true;
      else
      Status3b_1 = false;
      end
    state Part_Arrives
      entry:
      Status3b_2 = false;
      during:
      Control_70.C_75_ID_Delivery2;
      Sensors_70.O_70_SInductive;
      Sensors_70.O_70_SPart;
      Sensors_80.O_80_Arm_Mag;
      if Sensors_70.O_70_SPart && ...
      ((Sensors_70.O_70_SInductive && ...
      Control_70.C_75_ID_Delivery2) | ...
      (~Sensors_70.O_70_SInductive && ...
      ~Control_70.C_75_ID_Delivery2)) && ...
      ~Sensors_80.O_80_Arm_Mag
      Status3b_2 = true;
      else
      Status3b_2 =false;
      end
    state Elevator_Up
      entry:
      Status3b_3 = false;
      during:
      Actuators_70.F_72_Elev_Up;
      if Actuators_70.F_72_Elev_Up
      Status3b_3 = true
      else
      Status3b_3 = false
      end
    state Elevator_StartsMovingUp
      entry:
      Status3b_4 = false;
      during:
      Sensors_70.O_70_SInductive;
      if ~Sensors_70.O_70_SInductive
      Status3b_4 = true
      else
      Status3b_4 = false
      end
    state Elevator_MiddleUp
      entry:
      Status3b_5 = false;
      during:
      Sensors_70.O_70_SStation;
      if ~Sensors_70.O_70_SStation
      Status3b_5 = true
      else
      Status3b_5 = false
      end
    state Elevator_High_Identify_Part
      entry:
      Status3b_6 = false;
      during:
      MetalicPart;
      Control_70.C_75_ID_Delivery1;
      Control_70.C_75_ID_Delivery2;
      Sensors_70.O_70_SPart_Height;
      if MetalicPart && ...
      Control_70.C_75_ID_Delivery2 && ...
      ~Control_70.C_75_ID_Delivery1;
      Status3b_6 = true
      end
      if ~MetalicPart && ...
      Control_70.C_75_ID_Delivery1 && ...
      ((Sensors_70.O_70_SPart_Height && ...
      Control_70.C_75_ID_Delivery2) | ...
      (~Sensors_70.O_70_SPart_Height && ...
      ~Control_70.C_75_ID_Delivery2))
      Status3b_6=true
      end
    state CheckPart
      entry:
      Part_Equal = false;
      Part_Different = false;
      during:
      Control_70.C_75_ID_Delivery1;
      Control_70.C_75_ID_Delivery2;
      Control_70.C_75_RQ_Delivery1;
      Control_70.C_75_RQ_Delivery2;
      if (Control_70.C_75_ID_Delivery1 == ...
      Control_70.C_75_RQ_Delivery1) && ...
      (Control_70.C_75_ID_Delivery2 == ...
      Control_70.C_75_RQ_Delivery2)
      Part_Equal = true
      else
      Part_Different = true
      end
    state Pushes_Part
      entry:
      Status3b_7 = false;
      during:
      Actuators_70.F_72_Eject_Part;
      Actuators_70.F_72_Air_On;
      Sensors_70.O_70_SPart;
      if Actuators_70.F_72_Eject_Part && ...
      Actuators_70.F_72_Air_On && ...
      ~Sensors_70.O_70_SPart
      Status3b_7 = true
      else
      Status3b_7 = false
      end
    state Elevator_Down
      entry:
      Status3b_14 = false;
      during:
      AS_i_70.A_74_CRoute_Out;
      Actuators_70.F_72_Elev_Down;
      Control_70.C_75_Part_Del;
      if AS_i_70.A_74_CRoute_Out && ...
      ~Actuators_70.F_72_Elev_Down&& ...
      Control_70.C_75_Part_Del
      Status3b_14 = true
      else
      Status3b_14 = false
      end
    state Part_ArrivesAtCart
      entry:
      Status3b_9 = false;
      during:
      AS_i_70.A_74_Cart_Full;
      AS_i_70.A_74_Optic;
      Actuators_70.F_72_Air_On;
      Actuators_70.F_73_Led_Extra2
      if AS_i_70.A_74_Optic && ...
      AS_i_70.A_74_Cart_Full && ...
      ~Actuators_70.F_72_Air_On && ...
      Actuators_70.F_73_Led_Extra2;
      Status3b_9 = true
      else
      Status3b_9 = false
      end
    state End_Process
      entry:
      Status3b15 = false;
      during:
      AS_i_70.A_74_CRoute_Out;
      if  ~AS_i_70.A_74_CRoute_Out;
      Status3b_15 = true
      else
      Status3b_15 = false
      end
    state Metalic_Identify
      entry:
      MetalicPart = false;
      during:
      Sensors_70.O_70_SInductive;
      if Sensors_70.O_70_SInductive
      MetalicPart = true
      else
      MetalicPart = false
      end
    state Elevator_StartsMovingDown1
      entry:
      Status3b_16 = false;
      during:
      Actuators_70.F_72_Elev_Down;
      Actuators_70.F_72_Elev_Up;
      if Actuators_70.F_72_Elev_Down && ...
      ~Actuators_70.F_72_Elev_Up
      Status3b_16 = true
      else
      Status3b_16 = false
      end
    state Elevator_MiddleDown1
      entry:
      Status3b_17 = false;
      during:
      Sensors_70.O_70_SStation;
      if ~Sensors_70.O_70_SStation
      Status3b_17 = true
      else
      Status3b_17 = false
      end
    state Elevator_InductiveDown1
      entry:
      Status3b_18 = false;
      during:
      Sensors_70.O_70_SInductive;
      if ~Sensors_70.O_70_SInductive
      Status3b_18 = true
      else
      Status3b_18 = false
      end
    state Elevator_Down1
      entry:
      Status3b_19 = false;
      during:
      Actuators_70.F_72_Eject_Part
      Actuators_70.F_72_Elev_Down
      if Actuators_70.F_72_Eject_Part && ...
      ~Actuators_70.F_72_Elev_Down
      Status3b_19 = true
      else
      Status3b_19 = false
      end
    state Piston_Back1
      entry:
      Status3b_20 = false;
      during:
      Actuators_70.F_72_Eject_Part
      Sensors_70.O_70_Pist_Bck;
      Sensors_70.O_70_SPart
      Control_70.C_75_RQ_Wrong;
      if ~Actuators_70.F_72_Eject_Part && ...
      Sensors_70.O_70_Pist_Bck && ...
      ~Sensors_70.O_70_SPart && ...
      Control_70.C_75_RQ_Wrong;
      Status3b_20 = true
      else
      Status3b_20 = false
      end
    (default) -> Requested_Delivery.InitialCondition
    Requested_Delivery.Elevator_StartsMovingDown -> Requested_Delivery.Elevator_MiddleDown : [Status3b_11 == true && ...
        | Sensors_70.O_70_SStation == true]
    Requested_Delivery.Piston_Back -> Requested_Delivery.Elevator_StartsMovingDown : [Status3b_10 == true && ...
        | Sensors_70.O_70_Pist_Bck == true]
    Requested_Delivery.Elevator_MiddleDown -> Requested_Delivery.Elevator_InductiveDown : [Status3b_12 == true && ...
        | Sensors_70.O_70_SInductive == true]
    Requested_Delivery.Part_Arrives -> Requested_Delivery.Elevator_Up : [Status3b_2 == true && ...
        | Sensors_80.O_80_Arm_Mag == true ]
    Requested_Delivery.Pushes_Part -> Requested_Delivery.Part_HeightSensor : [Status3b_7 == true && ...
        | Sensors_70.O_70_Pist_Bck == false]
    Requested_Delivery.Elevator_Up -> Requested_Delivery.Elevator_StartsMovingUp : [Status3b_3 == true && ...
        | Sensors_70.O_70_SInductive == true ]
    Requested_Delivery.Elevator_StartsMovingUp -> Requested_Delivery.Elevator_MiddleUp : [Status3b_4 == true && ...
        | Sensors_70.O_70_SStation == true]
    Requested_Delivery.Elevator_MiddleUp -> Requested_Delivery.Elevator_High_Identify_Part : [Status3b_5 == true && ...
        | Sensors_70.O_70_Elev_High == true]
    Requested_Delivery.Elevator_InductiveDown -> Requested_Delivery.Elevator_Down : [St_RqDl_3a_13 == true && ...
        | Sensors_70.O_70_Elev_Low == true]
    Requested_Delivery.Part_HeightSensor -> (junction 1412)
    (junction 1412) -> Requested_Delivery.Piston_Back [order 1] : [Status3b_8 == true && ...
        | after (2,sec)]
    Requested_Delivery.Elevator_High_Identify_Part -> CheckPart : [Status3b_6 == true && ...
        | after (2,sec)]
    CheckPart -> (junction 1378)
    (junction 1378) -> Requested_Delivery.Pushes_Part [order 1] : [Part_Equal == true && ...
        | after (2,sec)]
    Requested_Delivery.InitialCondition -> (junction 1372) : [St_RqDl_3a_1 == true && ...
        | Sensors_70.O_70_SPart == true]
    (junction 1372) -> Requested_Delivery.Part_Arrives [order 1]
    (junction 1412) -> (junction 1410) [order 2] : [St_RqDl_3a_8 == true && ...
        | AS_i_70.A_74_Optic == true]
    (junction 1378) -> (junction 952) [order 2] : [Part_Different == true && ...
        | after (2,sec)]
    (junction 1372) -> (junction 1376) [order 2]
    Requested_Delivery.Elevator_Down -> Requested_Delivery.End_Process : after (2,sec)
    (junction 1410) -> Requested_Delivery.Part_ArrivesAtCart
    (junction 1376) -> Requested_Delivery.Metalic_Identify
    Elevator_MiddleDown1 -> Elevator_InductiveDown1 : [Status3b_17 == true && ...
        | Sensors_70.O_70_SInductive == true]
    Elevator_StartsMovingDown1 -> Elevator_MiddleDown1 : [Status3b_16 == true && ...
        | Sensors_70.O_70_SStation == true]
    Elevator_Down1 -> Piston_Back1 : [Status3b_19 == true && ...
        | Sensors_70.O_70_Pist_Bck == false]
    (junction 952) -> Elevator_StartsMovingDown1
    Elevator_InductiveDown1 -> Elevator_Down1 : [Status3b_18 == true && ...
        | Sensors_70.O_70_Elev_Low == true]
  state Distribution_Counted
    state ArmToMagazine1
      entry:
      St_DCd0_2c_14 = false;
      during:
      Actuators_80.F_82_Suction_Off;
      Actuators_80.F_82_Arm_2_Mag;
      Actuators_80.F_83_Led_Extra1;
      Control_80.C_85_Part_Del;
      if ~Actuators_80.F_82_Suction_Off && ...
      Actuators_80.F_82_Arm_2_Mag && ...
      Actuators_80.F_83_Led_Extra1 && ...
      Control_80.C_85_Part_Del
      St_DCd0_2c_14 = true;
      else
      St_DCd0_2c_14 = false;
      end
    state ArmCloseDeliver3
      entry:
      St_DCd0_2c_15 = false;
      during:
      Sensors_70.O_70_SStation;
      if Sensors_70.O_70_SStation
      St_DCd0_2c_15 = true;
      else
      St_DCd0_2c_15 = false;
      end
    state ArmArrives_Finish
      entry:
      St_DCd0_2c_16 = false;
      during:
      Actuators_80.F_82_Arm_2_Mag;
      if ~Actuators_80.F_82_Arm_2_Mag;
      St_DCd0_2c_16 = true;
      else
      St_DCd0_2c_16 = false;
      end
    state ArmToMagazine
      entry:
      St_DCd0_2c_8 = false;
      during:
      Actuators_80.F_82_Arm_2_Mag;
      if Actuators_80.F_82_Arm_2_Mag
      St_DCd0_2c_8 = true;
      else
      St_DCd0_2c_8 = false;
      end
    state ArmCloseDeliver1
      entry:
      St_DCd0_2c_9 = false;
      during:
      Sensors_70.O_70_SStation;
      if Sensors_70.O_70_SStation
      St_DCd0_2c_9 = true;
      else
      St_DCd0_2c_9 = false;
      end
    state ArmArrives_PicksPart
      entry:
      St_DCd0_2c_10 = false;
      during:
      Actuators_80.F_82_Suction_On;
      Actuators_80.F_82_Arm_2_Mag;
      if Actuators_80.F_82_Suction_On && ...
      ~Actuators_80.F_82_Arm_2_Mag
      St_DCd0_2c_10 = true;
      else
      St_DCd0_2c_10 = false;
      end
    state ArmToDelivery1
      entry:
      St_DCd0_2c_11 = false;
      during:
      Actuators_80.F_82_Arm_2_Del
      if Actuators_80.F_82_Arm_2_Del
      St_DCd0_2c_11 = true;
      else
      St_DCd0_2c_11 = false;
      end
    state ArmCloseDelivery2
      entry:
      St_DCd0_2c_12 = false;
      during:
      Sensors_70.O_70_SStation;
      if Sensors_70.O_70_SStation
      St_DCd0_2c_12 = true;
      else
      St_DCd0_2c_12 = false;
      end
    state ArmArrives_DeliversPart
      entry:
      St_DCd0_2c_13 = false;
      during:
      Actuators_80.F_82_Suction_On;
      Actuators_80.F_82_Suction_Off;
      Actuators_80.F_82_Arm_2_Del;
      if ~Actuators_80.F_82_Suction_On && ...
      Actuators_80.F_82_Suction_Off && ...
      ~Actuators_80.F_82_Arm_2_Del
      St_DCd0_2c_13 = true;
      else
      St_DCd0_2c_13 = false;
      end
    state PartDel_CheckLoop
      entry:
      LoopDistCont = false;
      during:
      Control_80.C_85_Part_Del
      Control_80.C_87_RQ_MParts
      if Control_80.C_85_Part_Del && ...
      Control_80.C_87_RQ_MParts == 0
      LoopDistCont = true;
      else
      LoopDistCont = false;
      end
    state InitialCondition
      entry:
      St_DCd0_2c_1 = false;
      during:
      Control_80.C_85_Initialization;
      Control_80.C_86_Mag_Parts;
      Control_80.C_82_Profibus;
      Control_80.C_85_Continuous;
      Sensors_80.O_80_Arm_Mag;
      Sensors_80.O_81_Key_Pos;
      if Control_80.C_85_Initialization&& ...
      Control_80.C_86_Mag_Parts ~= 0 && ...
      Control_80.C_82_Profibus && ...
      Control_80.C_85_Continuous && ...
      Sensors_80.O_80_Arm_Mag && ...
      Sensors_80.O_81_Key_Pos
      St_DCd0_2c_1 = true;
      else
      St_DCd0_2c_1 = false;
      end
    state ArmToDelivery
      entry:
      St_DCd0_2c_2 = false;
      during:
      Actuators_80.F_82_Arm_2_Del
      if Actuators_80.F_82_Arm_2_Del
      St_DCd0_2c_2 = true;
      else
      St_DCd0_2c_2 = false;
      end
    state ArmCloseDelivery
      entry:
      St_DCd0_2c_3 = false;
      during:
      Sensors_70.O_70_SStation;
      if Sensors_70.O_70_SStation
      St_DCd0_2c_3 = true;
      else
      St_DCd0_2c_3 = false;
      end
    state ArmArrives_FeedsPart
      entry:
      St_DCd0_2b_4 = false;
      during:
      Actuators_80.F_82_Pist_Adv;
      Actuators_80.F_82_Arm_2_Del;
      if Actuators_80.F_82_Pist_Adv && ...
      ~Actuators_80.F_82_Arm_2_Del
      St_DCd0_2b_4 = true;
      else
      St_DCd0_2b_4 = false;
      end
    state PistonStartsMoveForward
      entry:
      St_DCd0_2c_5 = false;
      during:
      Sensors_80.O_80_Pist_Bck;
      if ~Sensors_80.O_80_Pist_Bck
      St_DCd0_2c_5 = true;
      else
      St_DCd0_2c_5 = false;
      end
    state PartFed
      entry:
      St_DCd0_2c_6 = false;
      during:
      Actuators_80.F_82_Pist_Adv;
      if ~Actuators_80.F_82_Pist_Adv
      St_DCd0_2c_6 = true;
      else
      St_DCd0_2c_6 = false;
      end
    state PistonStartsMoveBackward
      entry:
      St_DCd0_2c_7 = false;
      during:
      Sensors_80.O_80_Pist_Fwd;
      if ~Sensors_80.O_80_Pist_Fwd
      St_DCd0_2c_7 = true;
      else
      St_DCd0_2c_7 = false;
      end
    state T1
      during:
      Control_80.C_85_Part_Del
      Actuators_80.F_83_Led_Extra1
    Distribution_Counted.InitialCondition -> Distribution_Counted.ArmToDelivery : [Sensors_80.O_81_Start == true | ...
        | Control_80.C_85_Start == true | ...
        | Control_70.C_75_RQ_Wrong == true | ...
        | (AS_i_70.A_74_CRoute_In80 == true && Sensors_80.O_81_Key_Pos == true) ]
    Distribution_Counted.ArmArrives_FeedsPart -> Distribution_Counted.PistonStartsMoveForward : [St_DCd0_2b_4 == true]
    Distribution_Counted.PartDel_CheckLoop -> Distribution_Counted.ArmToMagazine1 [order 2] : [LoopDistCont == false]
    Distribution_Counted.ArmCloseDeliver3 -> Distribution_Counted.ArmArrives_Finish : [Sensors_80.O_80_Arm_Mag == true && ...
        | St_DCd0_2c_15 == true]
    Distribution_Counted.ArmCloseDelivery2 -> Distribution_Counted.ArmArrives_DeliversPart : [Sensors_80.O_80_Arm_Del == true && ...
        | St_DCd0_2c_12 == true]
    Distribution_Counted.ArmCloseDelivery -> Distribution_Counted.ArmArrives_FeedsPart : [Sensors_80.O_80_Arm_Del == true && ...
        | St_DCd0_2c_3 == true]
    Distribution_Counted.PistonStartsMoveForward -> Distribution_Counted.PartFed : [Sensors_80.O_80_Pist_Fwd == true && ...
        | St_DCd0_2c_5 == true]
    Distribution_Counted.ArmArrives_DeliversPart -> Distribution_Counted.PartDel_CheckLoop : [Sensors_80.O_80_Part_Stuck == false && ...
        | St_DCd0_2c_13 == true]
    Distribution_Counted.ArmToMagazine1 -> Distribution_Counted.ArmCloseDeliver3 : [Sensors_80.O_80_Arm_Del == false &&...
        | St_DCd0_2c_14 == true]
    Distribution_Counted.ArmArrives_PicksPart -> Distribution_Counted.ArmToDelivery1 : [Sensors_80.O_80_Part_Stuck == true && ...
        | St_DCd0_2c_10 == true]
    Distribution_Counted.PistonStartsMoveBackward -> Distribution_Counted.ArmToMagazine : [Sensors_80.O_80_Pist_Bck == true && ...
        | St_DCd0_2c_7 == true]
    Distribution_Counted.ArmToDelivery -> Distribution_Counted.ArmCloseDelivery : [Sensors_80.O_80_Arm_Mag == false &&...
        | St_DCd0_2c_2 == true]
    Distribution_Counted.ArmToMagazine -> Distribution_Counted.ArmCloseDeliver1 : [Sensors_80.O_80_Arm_Del == false &&...
        | St_DCd0_2c_8 == true]
    Distribution_Counted.ArmCloseDeliver1 -> Distribution_Counted.ArmArrives_PicksPart : [Sensors_80.O_80_Arm_Mag == true && ...
        | St_DCd0_2c_9 == true]
    Distribution_Counted.PartFed -> Distribution_Counted.PistonStartsMoveBackward : [St_DCd0_2c_6 == true]
    (default) -> Distribution_Counted.InitialCondition
    Distribution_Counted.ArmToDelivery1 -> Distribution_Counted.ArmCloseDelivery2 : [Sensors_80.O_80_Arm_Mag == false &&...
        | St_DCd0_2c_11 == true]
    (junction 804) -> Distribution_Counted.ArmArrives_FeedsPart
    (junction 820) -> (junction 804)
    Distribution_Counted.PartDel_CheckLoop -> (junction 821) [order 1] : [LoopDistCont == true]
    Distribution_Counted.PartDel_CheckLoop -> Distribution_Counted.T1 [order 3] : after(4,sec)
    (junction 821) -> (junction 820)
  state RBS Output
    state STATE2
      entry:
      StatusRBS_1 = false;
      during:
      % Configuracao da estacao: so este bloco fica ativo se o bit dele estiver ligado
      if Control_60.C_65_Initialization && Control_60.C_65_RBS_Output
      StatusRBS_1 = true;
      else
      StatusRBS_1 = false;
      end
    state ESTATE7
      entry:
      StatusRBS_2 = false;
      during:
      % Janela de identificacao da peca (T1 = 2s no ladder)
      if Control_50.C_55_PD_Sort
      StatusRBS_2 = true;
      else
      StatusRBS_2 = false;
      end
    state ESTATE9
      entry:
      StatusRBS_3 = false;
      during:
      % Vermelha: SL1 avanca | Preta: SL2 avanca | Prata: ambas recuadas
      if ((Control_60.C_65_ID_1 && Control_60.C_65_ID_2) && Sensors_60.O_60_SL1_Fwd) || ...
      ((Control_60.C_65_ID_1 && ~Control_60.C_65_ID_2) && Sensors_60.O_60_SL2_Fwd) || ...
      ((~Control_60.C_65_ID_1 && Control_60.C_65_ID_2) && Sensors_60.O_60_SL1_Bck && Sensors_60.O_60_SL2_Bck)
      StatusRBS_3 = true;
      else
      StatusRBS_3 = false;
      end
    state ESTATE6
      entry:
      StatusRBS_4 = false;
      during:
      % Pino de identificacao acionado (LEITURA do CLP - sombra nao comanda)
      if Actuators_60.F_62_Identify
      StatusRBS_4 = true;
      else
      StatusRBS_4 = false;
      end
    state ESTATE8
      entry:
      StatusRBS_5 = false;
      during:
      % Pino recuado: ciclo concluido, pronto para a proxima peca
      if ~Actuators_60.F_62_Identify
      StatusRBS_5 = true;
      else
      StatusRBS_5 = false;
      end
    (default) -> STATE2
    ESTATE6 -> ESTATE8 : [Sensors_60.O_60_Part_Pass == true && StatusRBS_4 == true]
    ESTATE9 -> ESTATE6 : [StatusRBS_3 == true]
    STATE2 -> ESTATE7 : [Control_50.C_55_PD_Sort == true && Sensors_50.O_50_Claw_Del == true && StatusRBS_1 == true]
    ESTATE7 -> ESTATE9 : [(Control_60.C_65_ID_1 == true || Control_60.C_65_ID_2 == true || after(2, sec)) && StatusRBS_2 == true]
    ESTATE8 -> STATE2 : [StatusRBS_5 == true]
  note: Conveyor
  state CartToProcessing4
    state InitialCondition
      entry:
      St_C2P4_4_1 = false;
      during:
      Actuators_20.F_22_Conveyor;
      AS_i_70.A_74_Cart_Full;
      AS_i_70.A_73_TestCartID;
      AS_i_70.A_74_Pist_Bck;
      AS_i_70.A_74_Release_FB;
      if ~Actuators_20.F_22_Conveyor && ...
      AS_i_70.A_74_Cart_Full && ...
      ~AS_i_70.A_73_TestCartID ~= 0 && ...
      ~AS_i_70.A_74_Pist_Bck && ...
      ~AS_i_70.A_74_Release_FB
      St_C2P4_4_1 = true;
      else
      St_C2P4_4_1 = false;
      end
    state StartsProcess
      entry:
      St_C2P4_4_2 = false;
      during:
      Actuators_20.F_22_Conveyor;
      AS_i_70.A_73_TestCartID;
      AS_i_70.A_74_Pist_Bck;
      AS_i_70.A_74_Release_FB;
      if Actuators_20.F_22_Conveyor && ...
      AS_i_70.A_73_TestCartID == 0 && ...
      AS_i_70.A_74_Pist_Bck && ...
      AS_i_70.A_74_Release_FB
      St_C2P4_4_2 = true;
      else
      St_C2P4_4_2 = false;
      end
    state PartLeavesSensor
      entry:
      St_C2P4_4_3 = false;
      during:
      Actuators_70.F_73_Led_Extra2;
      AS_i_70.A_74_Cart_Full;
      AS_i_70.A_74_Optic;
      if ~Actuators_70.F_73_Led_Extra2 && ...
      ~AS_i_70.A_74_Cart_Full && ...
      ~AS_i_70.A_74_Optic
      St_C2P4_4_3 = true;
      else
      St_C2P4_4_3 = false;
      end
    state CartStartsMoving
      entry:
      St_C2P4_4_4 = false;
      during:
      Actuators_70.F_73_Led_Extra1;
      AS_i_70.A_74_No_Cart;
      AS_i_70.A_74_Cart_Stat;
      if Actuators_70.F_73_Led_Extra1 && ...
      AS_i_70.A_74_No_Cart && ...
      ~AS_i_70.A_74_Cart_Stat
      St_C2P4_4_4 = true;
      else
      St_C2P4_4_4 = false;
      end
    state CartGetsNearNextStation
      entry:
      St_C2P4_4_5 = false;
      during:
      AS_i_70.A_74_Cart_Next;
      AS_i_70.A_74_Pist_Bck;
      AS_i_70.A_74_Release_FB;
      if AS_i_70.A_74_Cart_Next && ...
      ~AS_i_70.A_74_Pist_Bck && ...
      ~AS_i_70.A_74_Release_FB
      St_C2P4_4_5 = true;
      else
      St_C2P4_4_5 = false;
      end
    state DetectionofCartNumberinStation
      entry:
      St_C2P4_4_6 = false;
      during:
      AS_i_90.A_93_ProcCartID
      if ~AS_i_90.A_93_ProcCartID ~=0
      St_C2P4_4_6 = true;
      else
      St_C2P4_4_6 = false;
      end
    state CartPassesNextStation
      entry:
      St_C2P4_4_7 = false;
      during:
      AS_i_70.A_74_Cart_Next
      if ~AS_i_70.A_74_Cart_Next
      St_C2P4_4_7 = true;
      else
      St_C2P4_4_7 = false;
      end
    state PartArrivesSensor
      entry:
      St_C2P4_4_8 = false;
      during:
      AS_i_90.A_94_Optic;
      if AS_i_90.A_94_Optic
      St_C2P4_4_8 = true;
      else
      St_C2P4_4_8 = false;
      end
    state CartArrivesinNextStation
      entry:
      St_C2P4_4_9 = false;
      during:
      Control_20.C_25_CartDel;
      Actuators_90.F_93_Led_Extra1;
      AS_i_90.A_94_Cart_Stat;
      AS_i_90.A_94_No_Cart;
      AS_i_90.A_94_Cart_Full;
      AS_i_90.A_94_CRoute_In;
      if Control_20.C_25_CartDel && ...
      ~Actuators_90.F_93_Led_Extra1 && ...
      AS_i_90.A_94_Cart_Stat && ...
      ~AS_i_90.A_94_No_Cart && ...
      AS_i_90.A_94_Cart_Full && ...
      AS_i_90.A_94_CRoute_In
      St_C2P4_4_9 = true;
      else
      St_C2P4_4_9 = false;
      end
    state T1
      during:
      Control_20.C_25_Request
    state T3
      during:
      Control_20.C_25_CartDel
    state T2
      during:
      AS_i_90.A_94_CRoute_In
    (default) -> CartToProcessing4.InitialCondition
    CartToProcessing4.DetectionofCartNumberinStation -> CartToProcessing4.CartPassesNextStation : [Sensors_20.O_24_Cart_Next == false && ...
        | St_C2P4_4_6 == true]
    CartToProcessing4.InitialCondition -> CartToProcessing4.StartsProcess : [Control_20.C_25_Request == true && ...
        |  St_C2P4_4_1 == true]
    CartToProcessing4.StartsProcess -> CartToProcessing4.PartLeavesSensor [order 1] : [Sensors_20.O_24_Optic == false && ...
        | St_C2P4_4_2 == true]
    CartToProcessing4.PartLeavesSensor -> CartToProcessing4.CartStartsMoving : [Sensors_20.O_24_Cart_Stat == false && ...
        | St_C2P4_4_3 == true]
    CartToProcessing4.CartStartsMoving -> CartToProcessing4.CartGetsNearNextStation : [Sensors_20.O_24_Cart_Next == true && ...
        | St_C2P4_4_4 == true]
    CartToProcessing4.CartGetsNearNextStation -> CartToProcessing4.DetectionofCartNumberinStation : [Sensors_20.O_24_Count == true && ...
        | St_C2P4_4_5 == true]
    CartToProcessing4.CartPassesNextStation -> CartToProcessing4.PartArrivesSensor : [Sensors_20.O_25_Optic == true && ...
        | St_C2P4_4_7 == true]
    CartToProcessing4.PartArrivesSensor -> CartToProcessing4.CartArrivesinNextStation : [Sensors_20.O_25_Cart_Stat == true && ...
        | St_C2P4_4_8 == true]
    CartToProcessing4.StartsProcess -> CartToProcessing4.T1 [order 2] : [after(2, sec)]
    CartToProcessing4.CartArrivesinNextStation -> (junction 2095)
    (junction 2095) -> CartToProcessing4.T3 [order 2] : [after(3,sec)]
    (junction 2095) -> CartToProcessing4.T2 [order 1] : [after(2,sec)]
  note: Conveyor
  note: Processing [100]
  state CartToProcessing
    state InitialCondition
      entry:
      St_C2P0_4_1 = false;
      during:
      Actuators_20.F_22_Conveyor;
      AS_i_70.A_74_Cart_Full;
      AS_i_70.A_73_TestCartID;
      AS_i_70.A_74_Pist_Bck;
      AS_i_70.A_74_Release_FB;
      if ~Actuators_20.F_22_Conveyor && ...
      AS_i_70.A_74_Cart_Full && ...
      ~AS_i_70.A_73_TestCartID ~= 0 && ...
      ~AS_i_70.A_74_Pist_Bck && ...
      ~AS_i_70.A_74_Release_FB
      St_C2P0_4_1 = true;
      else
      St_C2P0_4_1 = false;
      end
    state StartsProcess
      entry:
      St_C2P0_4_2 = false;
      during:
      Actuators_20.F_22_Conveyor;
      AS_i_70.A_73_TestCartID;
      AS_i_70.A_74_Pist_Bck;
      AS_i_70.A_74_Release_FB;
      if Actuators_20.F_22_Conveyor && ...
      AS_i_70.A_73_TestCartID == 0 && ...
      AS_i_70.A_74_Pist_Bck && ...
      AS_i_70.A_74_Release_FB
      St_C2P0_4_2 = true;
      else
      St_C2P0_4_2 = false;
      end
    state PartLeavesSensor
      entry:
      St_C2P0_4_3 = false;
      during:
      Actuators_70.F_73_Led_Extra2;
      AS_i_70.A_74_Cart_Full;
      AS_i_70.A_74_Optic;
      if ~Actuators_70.F_73_Led_Extra2 && ...
      ~AS_i_70.A_74_Cart_Full && ...
      ~AS_i_70.A_74_Optic
      St_C2P0_4_3 = true;
      else
      St_C2P0_4_3 = false;
      end
    state CartStartsMoving
      entry:
      St_C2P0_4_4 = false;
      during:
      Actuators_70.F_73_Led_Extra1;
      AS_i_70.A_74_No_Cart;
      AS_i_70.A_74_Cart_Stat;
      if Actuators_70.F_73_Led_Extra1 && ...
      AS_i_70.A_74_No_Cart && ...
      ~AS_i_70.A_74_Cart_Stat
      St_C2P0_4_4 = true;
      else
      St_C2P0_4_4 = false;
      end
    state CartGetsNearNextStation
      entry:
      St_C2P0_4_5 = false;
      during:
      AS_i_70.A_74_Cart_Next;
      AS_i_70.A_74_Pist_Bck;
      AS_i_70.A_74_Release_FB;
      if AS_i_70.A_74_Cart_Next && ...
      ~AS_i_70.A_74_Pist_Bck && ...
      ~AS_i_70.A_74_Release_FB
      St_C2P0_4_5 = true;
      else
      St_C2P0_4_5 = false;
      end
    state DetectionofCartNumberinStation
      entry:
      St_C2P0_4_6 = false;
      during:
      AS_i_90.A_93_ProcCartID
      if ~AS_i_90.A_93_ProcCartID ~=0
      St_C2P0_4_6 = true;
      else
      St_C2P0_4_6 = false;
      end
    state CartPassesNextStation
      entry:
      St_C2P0_4_7 = false;
      during:
      AS_i_70.A_74_Cart_Next
      if ~AS_i_70.A_74_Cart_Next
      St_C2P0_4_7 = true;
      else
      St_C2P0_4_7 = false;
      end
    state PartArrivesSensor
      entry:
      St_C2P0_4_8 = false;
      during:
      AS_i_90.A_94_Optic;
      if AS_i_90.A_94_Optic
      St_C2P0_4_8 = true;
      else
      St_C2P0_4_8 = false;
      end
    state CartArrivesinNextStation
      entry:
      St_C2P0_4_9 = false;
      during:
      Control_20.C_25_CartDel;
      Actuators_90.F_93_Led_Extra1;
      AS_i_90.A_94_Cart_Stat;
      AS_i_90.A_94_No_Cart;
      AS_i_90.A_94_Cart_Full;
      AS_i_90.A_94_CRoute_In;
      if Control_20.C_25_CartDel && ...
      ~Actuators_90.F_93_Led_Extra1 && ...
      AS_i_90.A_94_Cart_Stat && ...
      ~AS_i_90.A_94_No_Cart && ...
      AS_i_90.A_94_Cart_Full && ...
      AS_i_90.A_94_CRoute_In
      St_C2P0_4_9 = true;
      else
      St_C2P0_4_9 = false;
      end
    state T1
      during:
      Control_20.C_25_Request
    state T3
      during:
      Control_20.C_25_CartDel
    state T2
      during:
      AS_i_90.A_94_CRoute_In
    (default) -> CartToProcessing.InitialCondition
    CartToProcessing.DetectionofCartNumberinStation -> CartToProcessing.CartPassesNextStation : [Sensors_20.O_24_Cart_Next == false && ...
        | St_C2P0_4_6 == true]
    CartToProcessing.InitialCondition -> CartToProcessing.StartsProcess : [Control_20.C_25_Request == true && ...
        |  St_C2P0_4_1 == true]
    CartToProcessing.StartsProcess -> CartToProcessing.PartLeavesSensor [order 1] : [Sensors_20.O_24_Optic == false && ...
        | St_C2P0_4_2 == true]
    CartToProcessing.PartLeavesSensor -> CartToProcessing.CartStartsMoving : [Sensors_20.O_24_Cart_Stat == false && ...
        | St_C2P0_4_3 == true]
    CartToProcessing.CartStartsMoving -> CartToProcessing.CartGetsNearNextStation : [Sensors_20.O_24_Cart_Next == true && ...
        | St_C2P0_4_4 == true]
    CartToProcessing.CartGetsNearNextStation -> CartToProcessing.DetectionofCartNumberinStation : [Sensors_20.O_24_Count == true && ...
        | St_C2P0_4_5 == true]
    CartToProcessing.CartPassesNextStation -> CartToProcessing.PartArrivesSensor : [Sensors_20.O_25_Optic == true && ...
        | St_C2P0_4_7 == true]
    CartToProcessing.PartArrivesSensor -> CartToProcessing.CartArrivesinNextStation : [Sensors_20.O_25_Cart_Stat == true && ...
        | St_C2P0_4_8 == true]
    CartToProcessing.StartsProcess -> CartToProcessing.T1 [order 2] : [after(2, sec)]
    CartToProcessing.CartArrivesinNextStation -> (junction 1033)
    (junction 1033) -> CartToProcessing.T3 [order 2] : [after(3,sec)]
    (junction 1033) -> CartToProcessing.T2 [order 1] : [after(2,sec)]
  state RSB Output
    state STATE1
      entry:
      StatusRSB_1 = false;
      during:
      % Configuracao da estacao: so este bloco fica ativo se o bit dele estiver ligado
      if Control_60.C_65_Initialization && Control_60.C_65_RSB_Output
      StatusRSB_1 = true;
      else
      StatusRSB_1 = false;
      end
    state ESTATE2
      entry:
      StatusRSB_2 = false;
      during:
      % Janela de identificacao da peca (T1 = 2s no ladder)
      if Control_50.C_55_PD_Sort
      StatusRSB_2 = true;
      else
      StatusRSB_2 = false;
      end
    state ESTATE3
      entry:
      StatusRSB_3 = false;
      during:
      % Vermelha: SL1 avanca | Prata: SL2 avanca | Preta: ambas recuadas
      if ((Control_60.C_65_ID_1 && Control_60.C_65_ID_2) && Sensors_60.O_60_SL1_Fwd) || ...
      ((~Control_60.C_65_ID_1 && Control_60.C_65_ID_2) && Sensors_60.O_60_SL2_Fwd) || ...
      ((Control_60.C_65_ID_1 && ~Control_60.C_65_ID_2) && Sensors_60.O_60_SL1_Bck && Sensors_60.O_60_SL2_Bck)
      StatusRSB_3 = true;
      else
      StatusRSB_3 = false;
      end
    state ESTATE4
      entry:
      StatusRSB_4 = false;
      during:
      % Pino de identificacao acionado (LEITURA do CLP - sombra nao comanda)
      if Actuators_60.F_62_Identify
      StatusRSB_4 = true;
      else
      StatusRSB_4 = false;
      end
    state ESTATE5
      entry:
      StatusRSB_5 = false;
      during:
      % Pino recuado: ciclo concluido, pronto para a proxima peca
      if ~Actuators_60.F_62_Identify
      StatusRSB_5 = true;
      else
      StatusRSB_5 = false;
      end
    (default) -> RSB.STATE1
    RSB.ESTATE5 -> RSB.STATE1 : [StatusRSB_5 == true]
    RSB.ESTATE4 -> RSB.ESTATE5 : [Sensors_60.O_60_Part_Pass == true && StatusRSB_4 == true]
    RSB.ESTATE3 -> RSB.ESTATE4 : [StatusRSB_3 == true]
    RSB.ESTATE2 -> RSB.ESTATE3 : [(Control_60.C_65_ID_1 == true || Control_60.C_65_ID_2 == true || after(2, sec)) && StatusRSB_2 == true]
    RSB.STATE1 -> RSB.ESTATE2 : [Control_50.C_55_PD_Sort == true && Sensors_50.O_50_Claw_Del == true && StatusRSB_1 == true]
  state Processing_TestOnly
    state Config_TOnly
      entry:
      St_TOnly_1 = false;
      during:
      % FB4 Test Part Only - bloco ativo so neste modo
      if Control_100.C_105_Initialization && Control_100.C_105_Test
      St_TOnly_1 = true;
      else
      St_TOnly_1 = false;
      end
    state Aguarda_TOnly
      entry:
      St_TOnly_2 = false;
      during:
      % N1: condicoes para iniciar o ciclo de teste
      if Sensors_100.O_100_PInit_Pos && Sensors_90.O_90_Claw_High && Sensors_100.O_100_RT_Sensor && ~Actuators_100.F_102_RT_On
      St_TOnly_2 = true;
      else
      St_TOnly_2 = false;
      end
    state GiraTeste_TOnly
      entry:
      St_TOnly_3 = false;
      during:
      % N2: mesa girando ate a posicao de teste (contador C4, preset 4)
      if Actuators_100.F_102_RT_On
      St_TOnly_3 = true;
      else
      St_TOnly_3 = false;
      end
    state PosTeste_TOnly
      entry:
      St_TOnly_4 = false;
      during:
      % N3: peca na posicao de teste, temporizador de 2s
      if ~Actuators_100.F_102_RT_On && Sensors_100.O_100_PTest_Pos && Sensors_100.O_100_RT_Sensor
      St_TOnly_4 = true;
      else
      St_TOnly_4 = false;
      end
    state Retirada_TOnly
      entry:
      St_TOnly_7 = false;
      during:
      % N1(R): peca retirada pela garra da HD2, reseta o ciclo
      if Sensors_90.O_90_Claw_Del && Sensors_90.O_90_Claw_Low && Sensors_90.O_90_Part_in_Claw
      St_TOnly_7 = true;
      else
      St_TOnly_7 = false;
      end
    state Resultado_TOnly
      entry:
      St_TOnly_6 = false;
      during:
      % N5/N6: PTest_Ok define OK ou Falha (Profibus)
      if Control_100.C_105_Test_Ok || Control_100.C_105_Test_Fail
      St_TOnly_6 = true;
      else
      St_TOnly_6 = false;
      end
    state Testando_TOnly
      entry:
      St_TOnly_5 = false;
      during:
      % N4: pino de teste acionado
      if Actuators_100.F_102_Test_Pin
      St_TOnly_5 = true;
      else
      St_TOnly_5 = false;
      end
    Config_TOnly -> Aguarda_TOnly : [St_TOnly_1 == true]
    Aguarda_TOnly -> GiraTeste_TOnly : [St_TOnly_2 == true]
    GiraTeste_TOnly -> PosTeste_TOnly : [St_TOnly_3 == true]
    (default) -> Config_TOnly
    PosTeste_TOnly -> Testando_TOnly : [(St_TOnly_4 == true) && after(2, sec)]
    Testando_TOnly -> Resultado_TOnly : [St_TOnly_5 == true]
    Resultado_TOnly -> Retirada_TOnly : [St_TOnly_6 == true]
  note: Handling 2 [90]
  note: Storage [40]
  state Store Par
    state InitialCondition
      entry:
      St_Stor_5_1 = false;
      during:
      AS_i_90.A_94_Cart_Full;
      Control_90.C_95_Initialization;
      Control_90.C_95_Cart2Del;
      Control_90.C_92_Profibus;
      Sensors_90.O_91_Key_Pos;
      if AS_i_90.A_94_Cart_Full && ...
      Control_90.C_95_Initialization && ...
      Control_90.C_95_Cart2Del && ...
      Control_90.C_92_Profibus && ...
      Sensors_90.O_91_Key_Pos
      St_Stor_5_1 = true;
      else
      St_Stor_5_1 = false;
      end
    state FinishesProcess
      entry:
      St_Stor_5_13 = false;
      during:
      Control_90.C_95_PD_Proc;
      if Control_90.C_95_PD_Proc
      St_Stor_5_13 = true;
      else
      St_Stor_5_13 = false;
      end
    (default) -> Store.InitialCondition
    Store.InitialCondition -> ? : [AS_i_90.A_94_CRoute_In == true && ...
        |  St_Stor_5_1 == true]
  state PartToProcessing
    state FinishesProcess
      entry:
      St_P2P0_5_13 = false;
      during:
      Control_90.C_95_PD_Proc;
      if Control_90.C_95_PD_Proc
      St_P2P0_5_13 = true;
      else
      St_P2P0_5_13 = false;
      end
    state ClawBeginsAscend
      entry:
      St_P2P0_5_12 = false;
      during:
      Sensors_90.O_90_Part_in_Claw;
      if ~Sensors_90.O_90_Part_in_Claw
      St_P2P0_5_12 = true;
      else
      St_P2P0_5_12 = false;
      end
    state DeliversPart
      entry:
      St_P2P0_5_11 = false;
      during:
      Actuators_90.F_92_Claw_Down;
      Actuators_90.F_92_Close_Claw;
      if ~Actuators_90.F_92_Claw_Down && ...
      ~Actuators_90.F_92_Close_Claw
      St_P2P0_5_11 = true;
      else
      St_P2P0_5_11 = false;
      end
    state ClawDescent
      entry:
      St_P2P0_5_10 = false;
      during:
      Sensors_90.O_90_Claw_Low;
      Sensors_90.O_90_Claw_High;
      if Sensors_90.O_90_Claw_Low && ...
      ~Sensors_90.O_90_Claw_High
      St_P2P0_5_10 = true;
      else
      St_P2P0_5_10 = false;
      end
    state ArmArrives
      entry:
      St_P2P0_5_9 = false;
      during:
      Actuators_90.F_92_Claw_2_Del;
      Actuators_90.F_92_Claw_Down;
      if ~Actuators_90.F_92_Claw_2_Del && ...
      Actuators_90.F_92_Claw_Down
      St_P2P0_5_9 = true;
      else
      St_P2P0_5_9 = false;
      end
    state ArmPassesStorage
      entry:
      St_P2P0_5_8 = false;
      during:
      Sensors_90.O_90_Claw_Reserve;
      if ~Sensors_90.O_90_Claw_Reserve;
      St_P2P0_5_8 = true;
      else
      St_P2P0_5_8 = false;
      end
    state ArmStartsMovement
      entry:
      St_P2P0_5_7 = false;
      during:
      Sensors_90.O_90_Claw_Reserve;
      if Sensors_90.O_90_Claw_Reserve;
      St_P2P0_5_7 = true;
      else
      St_P2P0_5_7 = false;
      end
    state ClawFinishesAscend
      entry:
      St_P2P0_5_6 = false;
      during:
      Actuators_90.F_92_Claw_2_Del;
      if Actuators_90.F_92_Claw_2_Del
      St_P2P0_5_6 = true;
      else
      St_P2P0_5_6 = false;
      end
    state PartLeavesCart
      entry:
      St_P2P0_5_5 = false;
      during:
      AS_i_90.A_94_Cart_Full;
      if ~AS_i_90.A_94_Cart_Full
      St_P2P0_5_5 = true;
      else
      St_P2P0_5_5 = false;
      end
    state PartPickup_BeginsAscend
      entry:
      St_P2P0_5_4 = false;
      during:
      Actuators_90.F_92_Claw_Down;
      Sensors_90.O_90_Claw_Low;
      if ~Actuators_90.F_92_Claw_Down && ...
      ~Sensors_90.O_90_Claw_Low
      St_P2P0_5_4 = true;
      else
      St_P2P0_5_4 = false;
      end
    state ClawFinishesDescent
      entry:
      St_P2P0_5_3 = false;
      during:
      Actuators_90.F_92_Close_Claw;
      if Actuators_90.F_92_Close_Claw
      St_P2P0_5_3 = true;
      else
      St_P2P0_5_3 = false;
      end
    state ClawBeginsDescent
      entry:
      St_P2P0_5_2 = false;
      during:
      Actuators_90.F_92_Claw_Down;
      Control_90.C_95_PD_Proc;
      Control_90.C_95_PD_Cart;
      Sensors_90.O_90_Claw_High;
      if Actuators_90.F_92_Claw_Down && ...
      ~Control_90.C_95_PD_Proc && ...
      ~Control_90.C_95_PD_Cart && ...
      ~Sensors_90.O_90_Claw_High
      St_P2P0_5_2 = true;
      else
      St_P2P0_5_2 = false;
      end
    state InitialCondition
      entry:
      St_P2P0_5_1 = false;
      during:
      AS_i_90.A_94_Cart_Full;
      Control_90.C_95_Initialization;
      Control_90.C_95_Cart2Del;
      Control_90.C_92_Profibus;
      Sensors_90.O_91_Key_Pos;
      if AS_i_90.A_94_Cart_Full && ...
      Control_90.C_95_Initialization && ...
      Control_90.C_95_Cart2Del && ...
      Control_90.C_92_Profibus && ...
      Sensors_90.O_91_Key_Pos
      St_P2P0_5_1 = true;
      else
      St_P2P0_5_1 = false;
      end
    (default) -> PartToProcessing.InitialCondition
    PartToProcessing.ArmStartsMovement -> PartToProcessing.ArmPassesStorage : [Sensors_90.O_90_Claw_Reserve == false && ...
        | St_P2P0_5_7 == true]
    PartToProcessing.ClawBeginsAscend -> PartToProcessing.FinishesProcess : [Sensors_90.O_90_Claw_High == true && ...
        | St_P2P0_5_12 == true]
    PartToProcessing.DeliversPart -> PartToProcessing.ClawBeginsAscend : [Sensors_90.O_90_Claw_Low && ...
        | St_P2P0_5_11 == true]
    PartToProcessing.ArmArrives -> PartToProcessing.ClawDescent : [Sensors_90.O_90_Claw_High == false && ...
        | St_P2P0_5_9 == true]
    PartToProcessing.ClawFinishesAscend -> PartToProcessing.ArmStartsMovement : [Sensors_90.O_90_Claw_Cart == false && ...
        | St_P2P0_5_6 == true]
    PartToProcessing.ClawFinishesDescent -> PartToProcessing.PartPickup_BeginsAscend : [Sensors_90.O_90_Part_in_Claw == true && ...
        | St_P2P0_5_3 == true]
    PartToProcessing.PartLeavesCart -> PartToProcessing.ClawFinishesAscend : [Sensors_90.O_90_Claw_High == true && ...
        | St_P2P0_5_5 == true]
    PartToProcessing.PartPickup_BeginsAscend -> PartToProcessing.PartLeavesCart : [AS_i_90.A_94_Optic == false && ...
        | St_P2P0_5_4 == true]
    PartToProcessing.ClawDescent -> PartToProcessing.DeliversPart : [Sensors_100.O_100_PInit_Pos == true && ...
        | St_P2P0_5_10 == true]
    PartToProcessing.ClawBeginsDescent -> PartToProcessing.ClawFinishesDescent : [Sensors_90.O_90_Claw_Low == true && ...
        | St_P2P0_5_2 == true]
    PartToProcessing.InitialCondition -> PartToProcessing.ClawBeginsDescent : [AS_i_90.A_94_CRoute_In == true && ...
        |  St_P2P0_5_1 == true]
    PartToProcessing.ArmPassesStorage -> PartToProcessing.ArmArrives : [Sensors_90.O_90_Claw_Del == true && ...
        | St_P2P0_5_8 == true]
  state SRB Output
    state STATE1
      entry:
      StatusSRB_1 = false;
      during:
      % Configuracao da estacao: so este bloco fica ativo se o bit dele estiver ligado
      if Control_60.C_65_Initialization && Control_60.C_65_SRB_Output
      StatusSRB_1 = true;
      else
      StatusSRB_1 = false;
      end
    state ESTATE2
      entry:
      StatusSRB_2 = false;
      during:
      % Janela de identificacao da peca (T1 = 2s no ladder)
      if Control_50.C_55_PD_Sort
      StatusSRB_2 = true;
      else
      StatusSRB_2 = false;
      end
    state ESTATE3
      entry:
      StatusSRB_3 = false;
      during:
      % Prata: SL1 avanca | Vermelha: SL2 avanca | Preta: ambas recuadas
      if ((~Control_60.C_65_ID_1 && Control_60.C_65_ID_2) && Sensors_60.O_60_SL1_Fwd) || ...
      ((Control_60.C_65_ID_1 && Control_60.C_65_ID_2) && Sensors_60.O_60_SL2_Fwd) || ...
      ((Control_60.C_65_ID_1 && ~Control_60.C_65_ID_2) && Sensors_60.O_60_SL1_Bck && Sensors_60.O_60_SL2_Bck)
      StatusSRB_3 = true;
      else
      StatusSRB_3 = false;
      end
    state ESTATE4
      entry:
      StatusSRB_4 = false;
      during:
      % Pino de identificacao acionado (LEITURA do CLP - sombra nao comanda)
      if Actuators_60.F_62_Identify
      StatusSRB_4 = true;
      else
      StatusSRB_4 = false;
      end
    state ESTATE5
      entry:
      StatusSRB_5 = false;
      during:
      % Pino recuado: ciclo concluido, pronto para a proxima peca
      if ~Actuators_60.F_62_Identify
      StatusSRB_5 = true;
      else
      StatusSRB_5 = false;
      end
    (default) -> SRB.STATE1
    SRB.ESTATE5 -> SRB.STATE1 : [StatusSRB_5 == true]
    SRB.ESTATE4 -> SRB.ESTATE5 : [Sensors_60.O_60_Part_Pass == true && StatusSRB_4 == true]
    SRB.ESTATE3 -> SRB.ESTATE4 : [StatusSRB_3 == true]
    SRB.ESTATE2 -> SRB.ESTATE3 : [(Control_60.C_65_ID_1 == true || Control_60.C_65_ID_2 == true || after(2, sec)) && StatusSRB_2 == true]
    SRB.STATE1 -> SRB.ESTATE2 : [Control_50.C_55_PD_Sort == true && Sensors_50.O_50_Claw_Del == true && StatusSRB_1 == true]
  state Retrieve Part
    state FinishesProcess
      entry:
      St_Retr_5_13 = false;
      during:
      Control_90.C_95_PD_Proc;
      if Control_90.C_95_PD_Proc
      St_Retr_5_13 = true;
      else
      St_Retr_5_13 = false;
      end
    state InitialCondition
      entry:
      St_Retr_5_1 = false;
      during:
      AS_i_90.A_94_Cart_Full;
      Control_90.C_95_Initialization;
      Control_90.C_95_Cart2Del;
      Control_90.C_92_Profibus;
      Sensors_90.O_91_Key_Pos;
      if AS_i_90.A_94_Cart_Full && ...
      Control_90.C_95_Initialization && ...
      Control_90.C_95_Cart2Del && ...
      Control_90.C_92_Profibus && ...
      Sensors_90.O_91_Key_Pos
      St_Retr_5_1 = true;
      else
      St_Retr_5_1 = false;
      end
    (default) -> Retrieve.InitialCondition
    Retrieve.InitialCondition -> ? : [AS_i_90.A_94_CRoute_In == true && ...
        |  St_Retr_5_1 == true]
  state Processing_TestDrill
    state Config_TDrill
      entry:
      St_TDrill_1 = false;
      during:
      % FB5 Test + Drill - bloco ativo so neste modo
      if Control_100.C_105_Initialization && Control_100.C_105_TestDrill
      St_TDrill_1 = true;
      else
      St_TDrill_1 = false;
      end
    state Aguarda_TDrill
      entry:
      St_TDrill_2 = false;
      during:
      % N1: condicoes para iniciar teste+furacao
      if Sensors_100.O_100_PInit_Pos && Sensors_90.O_90_Claw_High && Sensors_100.O_100_RT_Sensor && ~Actuators_100.F_102_RT_On
      St_TDrill_2 = true;
      else
      St_TDrill_2 = false;
      end
    state GiraTeste_TDrill
      entry:
      St_TDrill_3 = false;
      during:
      % N2: mesa girando ate posicao de teste (C6, preset 4)
      if Actuators_100.F_102_RT_On
      St_TDrill_3 = true;
      else
      St_TDrill_3 = false;
      end
    state PosTeste_TDrill
      entry:
      St_TDrill_4 = false;
      during:
      % N3: peca na posicao de teste, temporizador de 2s
      if ~Actuators_100.F_102_RT_On && Sensors_100.O_100_PTest_Pos && Sensors_100.O_100_RT_Sensor
      St_TDrill_4 = true;
      else
      St_TDrill_4 = false;
      end
    state Testando_TDrill
      entry:
      St_TDrill_5 = false;
      during:
      % N4: pino de teste acionado
      if Actuators_100.F_102_Test_Pin
      St_TDrill_5 = true;
      else
      St_TDrill_5 = false;
      end
    state Resultado_TDrill
      entry:
      St_TDrill_6 = false;
      during:
      % N5/N6: resultado do teste no Profibus
      if Control_100.C_105_Test_Ok || Control_100.C_105_Test_Fail
      St_TDrill_6 = true;
      else
      St_TDrill_6 = false;
      end
    state Retirada_TDrill
      entry:
      St_TDrill_11 = false;
      during:
      % N16: peca retirada pela garra da HD2, reseta o ciclo
      if Sensors_90.O_90_Claw_Del && Sensors_90.O_90_Claw_Low && Sensors_90.O_90_Part_in_Claw
      St_TDrill_11 = true;
      else
      St_TDrill_11 = false;
      end
    state GiraEntrega_TDrill
      entry:
      St_TDrill_10 = false;
      during:
      % N13/N14/N15: gira ate a entrega (C8 se OK, C9 se falha) e libera a peca
      if ~Actuators_100.F_102_RT_On && Sensors_100.O_100_PInit_Pos
      St_TDrill_10 = true;
      else
      St_TDrill_10 = false;
      end
    state Furando_TDrill
      entry:
      St_TDrill_9 = false;
      during:
      % N10/N11/N12: fura, sobe e libera o pino
      if Actuators_100.F_102_Drill_On || (Actuators_100.F_102_Drill_Up && Sensors_100.O_100_SDrill_High)
      St_TDrill_9 = true;
      else
      St_TDrill_9 = false;
      end
    state DesceFuro_TDrill
      entry:
      St_TDrill_8 = false;
      during:
      % N8/N9: trava a peca e desce a furadeira ate o fim de curso
      if Actuators_100.F_102_Drill_Pin && Actuators_100.F_102_Drill_Down && Sensors_100.O_100_SDrill_Low
      St_TDrill_8 = true;
      else
      St_TDrill_8 = false;
      end
    state GiraFuro_TDrill
      entry:
      St_TDrill_7 = false;
      during:
      % N7: so gira ate a furadeira se o teste passou (C7, preset 1)
      if Control_100.C_105_Test_Ok && Actuators_100.F_102_RT_On
      St_TDrill_7 = true;
      else
      St_TDrill_7 = false;
      end
    Config_TDrill -> Aguarda_TDrill : [St_TDrill_1 == true]
    Aguarda_TDrill -> GiraTeste_TDrill : [St_TDrill_2 == true]
    GiraTeste_TDrill -> PosTeste_TDrill : [St_TDrill_3 == true]
    PosTeste_TDrill -> Testando_TDrill : [(St_TDrill_4 == true) && after(2, sec)]
    Testando_TDrill -> Resultado_TDrill : [St_TDrill_5 == true]
    (default) -> Config_TDrill
    (junction 1856) -> (junction 1858)
    Resultado_TDrill -> GiraFuro_TDrill : [St_TDrill_6 == true]
    GiraFuro_TDrill -> DesceFuro_TDrill : [St_TDrill_7 == true]
    DesceFuro_TDrill -> Furando_TDrill : [St_TDrill_8 == true]
    Furando_TDrill -> GiraEntrega_TDrill : [St_TDrill_9 == true]
    GiraEntrega_TDrill -> Retirada_TDrill : [St_TDrill_10 == true]
  state PartToProcessing1
    state FinishesProcess
      entry:
      St_P2P1_5_13 = false;
      during:
      Control_90.C_95_PD_Proc;
      if Control_90.C_95_PD_Proc
      St_P2P1_5_13 = true;
      else
      St_P2P1_5_13 = false;
      end
    state ClawBeginsAscend
      entry:
      St_P2P1_5_12 = false;
      during:
      Sensors_90.O_90_Part_in_Claw;
      if ~Sensors_90.O_90_Part_in_Claw
      St_P2P1_5_12 = true;
      else
      St_P2P1_5_12 = false;
      end
    state DeliversPart
      entry:
      St_P2P1_5_11 = false;
      during:
      Actuators_90.F_92_Claw_Down;
      Actuators_90.F_92_Close_Claw;
      if ~Actuators_90.F_92_Claw_Down && ...
      ~Actuators_90.F_92_Close_Claw
      St_P2P1_5_11 = true;
      else
      St_P2P1_5_11 = false;
      end
    state ClawDescent
      entry:
      St_P2P1_5_10 = false;
      during:
      Sensors_90.O_90_Claw_Low;
      Sensors_90.O_90_Claw_High;
      if Sensors_90.O_90_Claw_Low && ...
      ~Sensors_90.O_90_Claw_High
      St_P2P1_5_10 = true;
      else
      St_P2P1_5_10 = false;
      end
    state ArmArrives
      entry:
      St_P2P1_5_9 = false;
      during:
      Actuators_90.F_92_Claw_2_Del;
      Actuators_90.F_92_Claw_Down;
      if ~Actuators_90.F_92_Claw_2_Del && ...
      Actuators_90.F_92_Claw_Down
      St_P2P1_5_9 = true;
      else
      St_P2P1_5_9 = false;
      end
    state ArmPassesStorage
      entry:
      St_P2P1_5_8 = false;
      during:
      Sensors_90.O_90_Claw_Reserve;
      if ~Sensors_90.O_90_Claw_Reserve;
      St_P2P1_5_8 = true;
      else
      St_P2P1_5_8 = false;
      end
    state ArmStartsMovement
      entry:
      St_P2P1_5_7 = false;
      during:
      Sensors_90.O_90_Claw_Reserve;
      if Sensors_90.O_90_Claw_Reserve;
      St_P2P1_5_7 = true;
      else
      St_P2P1_5_7 = false;
      end
    state ClawFinishesAscend
      entry:
      St_P2P1_5_6 = false;
      during:
      Actuators_90.F_92_Claw_2_Del;
      if Actuators_90.F_92_Claw_2_Del
      St_P2P1_5_6 = true;
      else
      St_P2P1_5_6 = false;
      end
    state PartLeavesCart
      entry:
      St_P2P1_5_5 = false;
      during:
      AS_i_90.A_94_Cart_Full;
      if ~AS_i_90.A_94_Cart_Full
      St_P2P1_5_5 = true;
      else
      St_P2P1_5_5 = false;
      end
    state PartPickup_BeginsAscend
      entry:
      St_P2P1_5_4 = false;
      during:
      Actuators_90.F_92_Claw_Down;
      Sensors_90.O_90_Claw_Low;
      if ~Actuators_90.F_92_Claw_Down && ...
      ~Sensors_90.O_90_Claw_Low
      St_P2P1_5_4 = true;
      else
      St_P2P1_5_4 = false;
      end
    state ClawFinishesDescent
      entry:
      St_P2P1_5_3 = false;
      during:
      Actuators_90.F_92_Close_Claw;
      if Actuators_90.F_92_Close_Claw
      St_P2P1_5_3 = true;
      else
      St_P2P1_5_3 = false;
      end
    state ClawBeginsDescent
      entry:
      St_P2P1_5_2 = false;
      during:
      Actuators_90.F_92_Claw_Down;
      Control_90.C_95_PD_Proc;
      Control_90.C_95_PD_Cart;
      Sensors_90.O_90_Claw_High;
      if Actuators_90.F_92_Claw_Down && ...
      ~Control_90.C_95_PD_Proc && ...
      ~Control_90.C_95_PD_Cart && ...
      ~Sensors_90.O_90_Claw_High
      St_P2P1_5_2 = true;
      else
      St_P2P1_5_2 = false;
      end
    state InitialCondition
      entry:
      St_P2P1_5_1 = false;
      during:
      AS_i_90.A_94_Cart_Full;
      Control_90.C_95_Initialization;
      Control_90.C_95_Cart2Del;
      Control_90.C_92_Profibus;
      Sensors_90.O_91_Key_Pos;
      if AS_i_90.A_94_Cart_Full && ...
      Control_90.C_95_Initialization && ...
      Control_90.C_95_Cart2Del && ...
      Control_90.C_92_Profibus && ...
      Sensors_90.O_91_Key_Pos
      St_P2P1_5_1 = true;
      else
      St_P2P1_5_1 = false;
      end
    (default) -> ? [order 2] : [Sensors_90.O_90_Claw_High == true && ...
        | St_P2P1_5_5 == true]
    (default) -> PartToProcessing1.InitialCondition [order 1]
    PartToProcessing1.ArmStartsMovement -> PartToProcessing1.ArmPassesStorage : [Sensors_90.O_90_Claw_Reserve == false && ...
        | St_P2P1_5_7 == true]
    PartToProcessing1.ClawBeginsAscend -> PartToProcessing1.FinishesProcess : [Sensors_90.O_90_Claw_High == true && ...
        | St_P2P1_5_12 == true]
    PartToProcessing1.DeliversPart -> PartToProcessing1.ClawBeginsAscend : [Sensors_90.O_90_Claw_Low && ...
        | St_P2P1_5_11 == true]
    PartToProcessing1.ArmArrives -> PartToProcessing1.ClawDescent : [Sensors_90.O_90_Claw_High == false && ...
        | St_P2P1_5_9 == true]
    PartToProcessing1.ClawFinishesAscend -> PartToProcessing1.ArmStartsMovement : [Sensors_90.O_90_Claw_Cart == false && ...
        | St_P2P1_5_6 == true]
    PartToProcessing1.ClawFinishesDescent -> PartToProcessing1.PartPickup_BeginsAscend : [Sensors_90.O_90_Part_in_Claw == true && ...
        | St_P2P1_5_3 == true]
    PartToProcessing1.PartLeavesCart -> PartToProcessing1.ClawFinishesAscend : [Sensors_90.O_90_Claw_High == true && ...
        | St_P2P1_5_5 == true]
    PartToProcessing1.PartPickup_BeginsAscend -> PartToProcessing1.PartLeavesCart : [AS_i_90.A_94_Optic == false && ...
        | St_P2P1_5_4 == true]
    PartToProcessing1.ClawDescent -> PartToProcessing1.DeliversPart : [Sensors_100.O_100_PInit_Pos == true && ...
        | St_P2P1_5_10 == true]
    PartToProcessing1.ClawBeginsDescent -> PartToProcessing1.ClawFinishesDescent : [Sensors_90.O_90_Claw_Low == true && ...
        | St_P2P1_5_2 == true]
    PartToProcessing1.InitialCondition -> PartToProcessing1.ClawBeginsDescent : [AS_i_90.A_94_CRoute_In == true && ...
        |  St_P2P1_5_1 == true]
    PartToProcessing1.ArmPassesStorage -> PartToProcessing1.ArmArrives : [Sensors_90.O_90_Claw_Del == true && ...
        | St_P2P1_5_8 == true]
  note: Conveyor
  note: Conveyor
  state CartToProcessing3
    state InitialCondition
      entry:
      St_C2P3_4_1 = false;
      during:
      Actuators_20.F_22_Conveyor;
      AS_i_70.A_74_Cart_Full;
      AS_i_70.A_73_TestCartID;
      AS_i_70.A_74_Pist_Bck;
      AS_i_70.A_74_Release_FB;
      if ~Actuators_20.F_22_Conveyor && ...
      AS_i_70.A_74_Cart_Full && ...
      ~AS_i_70.A_73_TestCartID ~= 0 && ...
      ~AS_i_70.A_74_Pist_Bck && ...
      ~AS_i_70.A_74_Release_FB
      St_C2P3_4_1 = true;
      else
      St_C2P3_4_1 = false;
      end
    state StartsProcess
      entry:
      St_C2P3_4_2 = false;
      during:
      Actuators_20.F_22_Conveyor;
      AS_i_70.A_73_TestCartID;
      AS_i_70.A_74_Pist_Bck;
      AS_i_70.A_74_Release_FB;
      if Actuators_20.F_22_Conveyor && ...
      AS_i_70.A_73_TestCartID == 0 && ...
      AS_i_70.A_74_Pist_Bck && ...
      AS_i_70.A_74_Release_FB
      St_C2P3_4_2 = true;
      else
      St_C2P3_4_2 = false;
      end
    state PartLeavesSensor
      entry:
      St_C2P3_4_3 = false;
      during:
      Actuators_70.F_73_Led_Extra2;
      AS_i_70.A_74_Cart_Full;
      AS_i_70.A_74_Optic;
      if ~Actuators_70.F_73_Led_Extra2 && ...
      ~AS_i_70.A_74_Cart_Full && ...
      ~AS_i_70.A_74_Optic
      St_C2P3_4_3 = true;
      else
      St_C2P3_4_3 = false;
      end
    state CartStartsMoving
      entry:
      St_C2P3_4_4 = false;
      during:
      Actuators_70.F_73_Led_Extra1;
      AS_i_70.A_74_No_Cart;
      AS_i_70.A_74_Cart_Stat;
      if Actuators_70.F_73_Led_Extra1 && ...
      AS_i_70.A_74_No_Cart && ...
      ~AS_i_70.A_74_Cart_Stat
      St_C2P3_4_4 = true;
      else
      St_C2P3_4_4 = false;
      end
    state CartGetsNearNextStation
      entry:
      St_C2P3_4_5 = false;
      during:
      AS_i_70.A_74_Cart_Next;
      AS_i_70.A_74_Pist_Bck;
      AS_i_70.A_74_Release_FB;
      if AS_i_70.A_74_Cart_Next && ...
      ~AS_i_70.A_74_Pist_Bck && ...
      ~AS_i_70.A_74_Release_FB
      St_C2P3_4_5 = true;
      else
      St_C2P3_4_5 = false;
      end
    state DetectionofCartNumberinStation
      entry:
      St_C2P3_4_6 = false;
      during:
      AS_i_90.A_93_ProcCartID
      if ~AS_i_90.A_93_ProcCartID ~=0
      St_C2P3_4_6 = true;
      else
      St_C2P3_4_6 = false;
      end
    state CartPassesNextStation
      entry:
      St_C2P3_4_7 = false;
      during:
      AS_i_70.A_74_Cart_Next
      if ~AS_i_70.A_74_Cart_Next
      St_C2P3_4_7 = true;
      else
      St_C2P3_4_7 = false;
      end
    state PartArrivesSensor
      entry:
      St_C2P3_4_8 = false;
      during:
      AS_i_90.A_94_Optic;
      if AS_i_90.A_94_Optic
      St_C2P3_4_8 = true;
      else
      St_C2P3_4_8 = false;
      end
    state CartArrivesinNextStation
      entry:
      St_C2P3_4_9 = false;
      during:
      Control_20.C_25_CartDel;
      Actuators_90.F_93_Led_Extra1;
      AS_i_90.A_94_Cart_Stat;
      AS_i_90.A_94_No_Cart;
      AS_i_90.A_94_Cart_Full;
      AS_i_90.A_94_CRoute_In;
      if Control_20.C_25_CartDel && ...
      ~Actuators_90.F_93_Led_Extra1 && ...
      AS_i_90.A_94_Cart_Stat && ...
      ~AS_i_90.A_94_No_Cart && ...
      AS_i_90.A_94_Cart_Full && ...
      AS_i_90.A_94_CRoute_In
      St_C2P3_4_9 = true;
      else
      St_C2P3_4_9 = false;
      end
    state T1
      during:
      Control_20.C_25_Request
    state T3
      during:
      Control_20.C_25_CartDel
    state T2
      during:
      AS_i_90.A_94_CRoute_In
    (default) -> CartToProcessing3.InitialCondition
    CartToProcessing3.DetectionofCartNumberinStation -> CartToProcessing3.CartPassesNextStation : [Sensors_20.O_24_Cart_Next == false && ...
        | St_C2P3_4_6 == true]
    CartToProcessing3.InitialCondition -> CartToProcessing3.StartsProcess : [Control_20.C_25_Request == true && ...
        |  St_C2P3_4_1 == true]
    CartToProcessing3.StartsProcess -> CartToProcessing3.PartLeavesSensor [order 1] : [Sensors_20.O_24_Optic == false && ...
        | St_C2P3_4_2 == true]
    CartToProcessing3.PartLeavesSensor -> CartToProcessing3.CartStartsMoving : [Sensors_20.O_24_Cart_Stat == false && ...
        | St_C2P3_4_3 == true]
    CartToProcessing3.CartStartsMoving -> CartToProcessing3.CartGetsNearNextStation : [Sensors_20.O_24_Cart_Next == true && ...
        | St_C2P3_4_4 == true]
    CartToProcessing3.CartGetsNearNextStation -> CartToProcessing3.DetectionofCartNumberinStation : [Sensors_20.O_24_Count == true && ...
        | St_C2P3_4_5 == true]
    CartToProcessing3.CartPassesNextStation -> CartToProcessing3.PartArrivesSensor : [Sensors_20.O_25_Optic == true && ...
        | St_C2P3_4_7 == true]
    CartToProcessing3.PartArrivesSensor -> CartToProcessing3.CartArrivesinNextStation : [Sensors_20.O_25_Cart_Stat == true && ...
        | St_C2P3_4_8 == true]
    CartToProcessing3.StartsProcess -> CartToProcessing3.T1 [order 2] : [after(2, sec)]
    CartToProcessing3.CartArrivesinNextStation -> (junction 1998)
    (junction 1998) -> CartToProcessing3.T3 [order 2] : [after(3,sec)]
    (junction 1998) -> CartToProcessing3.T2 [order 1] : [after(2,sec)]
  state CartToProcessing1
    state InitialCondition
      entry:
      St_C2P1_4_1 = false;
      during:
      Actuators_20.F_22_Conveyor;
      AS_i_70.A_74_Cart_Full;
      AS_i_70.A_73_TestCartID;
      AS_i_70.A_74_Pist_Bck;
      AS_i_70.A_74_Release_FB;
      if ~Actuators_20.F_22_Conveyor && ...
      AS_i_70.A_74_Cart_Full && ...
      ~AS_i_70.A_73_TestCartID ~= 0 && ...
      ~AS_i_70.A_74_Pist_Bck && ...
      ~AS_i_70.A_74_Release_FB
      St_C2P1_4_1 = true;
      else
      St_C2P1_4_1 = false;
      end
    state StartsProcess
      entry:
      St_C2P1_4_2 = false;
      during:
      Actuators_20.F_22_Conveyor;
      AS_i_70.A_73_TestCartID;
      AS_i_70.A_74_Pist_Bck;
      AS_i_70.A_74_Release_FB;
      if Actuators_20.F_22_Conveyor && ...
      AS_i_70.A_73_TestCartID == 0 && ...
      AS_i_70.A_74_Pist_Bck && ...
      AS_i_70.A_74_Release_FB
      St_C2P1_4_2 = true;
      else
      St_C2P1_4_2 = false;
      end
    state PartLeavesSensor
      entry:
      St_C2P1_4_3 = false;
      during:
      Actuators_70.F_73_Led_Extra2;
      AS_i_70.A_74_Cart_Full;
      AS_i_70.A_74_Optic;
      if ~Actuators_70.F_73_Led_Extra2 && ...
      ~AS_i_70.A_74_Cart_Full && ...
      ~AS_i_70.A_74_Optic
      St_C2P1_4_3 = true;
      else
      St_C2P1_4_3 = false;
      end
    state CartStartsMoving
      entry:
      St_C2P1_4_4 = false;
      during:
      Actuators_70.F_73_Led_Extra1;
      AS_i_70.A_74_No_Cart;
      AS_i_70.A_74_Cart_Stat;
      if Actuators_70.F_73_Led_Extra1 && ...
      AS_i_70.A_74_No_Cart && ...
      ~AS_i_70.A_74_Cart_Stat
      St_C2P1_4_4 = true;
      else
      St_C2P1_4_4 = false;
      end
    state CartGetsNearNextStation
      entry:
      St_C2P1_4_5 = false;
      during:
      AS_i_70.A_74_Cart_Next;
      AS_i_70.A_74_Pist_Bck;
      AS_i_70.A_74_Release_FB;
      if AS_i_70.A_74_Cart_Next && ...
      ~AS_i_70.A_74_Pist_Bck && ...
      ~AS_i_70.A_74_Release_FB
      St_C2P1_4_5 = true;
      else
      St_C2P1_4_5 = false;
      end
    state DetectionofCartNumberinStation
      entry:
      St_C2P1_4_6 = false;
      during:
      AS_i_90.A_93_ProcCartID
      if ~AS_i_90.A_93_ProcCartID ~=0
      St_C2P1_4_6 = true;
      else
      St_C2P1_4_6 = false;
      end
    state CartPassesNextStation
      entry:
      St_C2P1_4_7 = false;
      during:
      AS_i_70.A_74_Cart_Next
      if ~AS_i_70.A_74_Cart_Next
      St_C2P1_4_7 = true;
      else
      St_C2P1_4_7 = false;
      end
    state PartArrivesSensor
      entry:
      St_C2P1_4_8 = false;
      during:
      AS_i_90.A_94_Optic;
      if AS_i_90.A_94_Optic
      St_C2P1_4_8 = true;
      else
      St_C2P1_4_8 = false;
      end
    state CartArrivesinNextStation
      entry:
      St_C2P1_4_9 = false;
      during:
      Control_20.C_25_CartDel;
      Actuators_90.F_93_Led_Extra1;
      AS_i_90.A_94_Cart_Stat;
      AS_i_90.A_94_No_Cart;
      AS_i_90.A_94_Cart_Full;
      AS_i_90.A_94_CRoute_In;
      if Control_20.C_25_CartDel && ...
      ~Actuators_90.F_93_Led_Extra1 && ...
      AS_i_90.A_94_Cart_Stat && ...
      ~AS_i_90.A_94_No_Cart && ...
      AS_i_90.A_94_Cart_Full && ...
      AS_i_90.A_94_CRoute_In
      St_C2P1_4_9 = true;
      else
      St_C2P1_4_9 = false;
      end
    state T1
      during:
      Control_20.C_25_Request
    state T3
      during:
      Control_20.C_25_CartDel
    state T2
      during:
      AS_i_90.A_94_CRoute_In
    (default) -> CartToProcessing1.InitialCondition
    CartToProcessing1.DetectionofCartNumberinStation -> CartToProcessing1.CartPassesNextStation : [Sensors_20.O_24_Cart_Next == false && ...
        | St_C2P1_4_6 == true]
    CartToProcessing1.InitialCondition -> CartToProcessing1.StartsProcess : [Control_20.C_25_Request == true && ...
        |  St_C2P1_4_1 == true]
    CartToProcessing1.StartsProcess -> CartToProcessing1.PartLeavesSensor [order 1] : [Sensors_20.O_24_Optic == false && ...
        | St_C2P1_4_2 == true]
    CartToProcessing1.PartLeavesSensor -> CartToProcessing1.CartStartsMoving : [Sensors_20.O_24_Cart_Stat == false && ...
        | St_C2P1_4_3 == true]
    CartToProcessing1.CartStartsMoving -> CartToProcessing1.CartGetsNearNextStation : [Sensors_20.O_24_Cart_Next == true && ...
        | St_C2P1_4_4 == true]
    CartToProcessing1.CartGetsNearNextStation -> CartToProcessing1.DetectionofCartNumberinStation : [Sensors_20.O_24_Count == true && ...
        | St_C2P1_4_5 == true]
    CartToProcessing1.CartPassesNextStation -> CartToProcessing1.PartArrivesSensor : [Sensors_20.O_25_Optic == true && ...
        | St_C2P1_4_7 == true]
    CartToProcessing1.PartArrivesSensor -> CartToProcessing1.CartArrivesinNextStation : [Sensors_20.O_25_Cart_Stat == true && ...
        | St_C2P1_4_8 == true]
    CartToProcessing1.StartsProcess -> CartToProcessing1.T1 [order 2] : [after(2, sec)]
    CartToProcessing1.CartArrivesinNextStation -> (junction 1660)
    (junction 1660) -> CartToProcessing1.T3 [order 2] : [after(3,sec)]
    (junction 1660) -> CartToProcessing1.T2 [order 1] : [after(2,sec)]
  state SBR Output
    state STATE1
      entry:
      StatusSBR_1 = false;
      during:
      % Configuracao da estacao: so este bloco fica ativo se o bit dele estiver ligado
      if Control_60.C_65_Initialization && Control_60.C_65_SBR_Output
      StatusSBR_1 = true;
      else
      StatusSBR_1 = false;
      end
    state ESTATE2
      entry:
      StatusSBR_2 = false;
      during:
      % Janela de identificacao da peca (T1 = 2s no ladder)
      if Control_50.C_55_PD_Sort
      StatusSBR_2 = true;
      else
      StatusSBR_2 = false;
      end
    state ESTATE3
      entry:
      StatusSBR_3 = false;
      during:
      % Prata: SL1 avanca | Preta: SL2 avanca | Vermelha: ambas recuadas
      if ((~Control_60.C_65_ID_1 && Control_60.C_65_ID_2) && Sensors_60.O_60_SL1_Fwd) || ...
      ((Control_60.C_65_ID_1 && ~Control_60.C_65_ID_2) && Sensors_60.O_60_SL2_Fwd) || ...
      ((Control_60.C_65_ID_1 && Control_60.C_65_ID_2) && Sensors_60.O_60_SL1_Bck && Sensors_60.O_60_SL2_Bck)
      StatusSBR_3 = true;
      else
      StatusSBR_3 = false;
      end
    state ESTATE4
      entry:
      StatusSBR_4 = false;
      during:
      % Pino de identificacao acionado (LEITURA do CLP - sombra nao comanda)
      if Actuators_60.F_62_Identify
      StatusSBR_4 = true;
      else
      StatusSBR_4 = false;
      end
    state ESTATE5
      entry:
      StatusSBR_5 = false;
      during:
      % Pino recuado: ciclo concluido, pronto para a proxima peca
      if ~Actuators_60.F_62_Identify
      StatusSBR_5 = true;
      else
      StatusSBR_5 = false;
      end
    (default) -> SBR.STATE1
    SBR.ESTATE2 -> SBR.ESTATE3 : [(Control_60.C_65_ID_1 == true || Control_60.C_65_ID_2 == true || after(2, sec)) && StatusSBR_2 == true]
    SBR.ESTATE4 -> SBR.ESTATE5 : [Sensors_60.O_60_Part_Pass == true && StatusSBR_4 == true]
    SBR.ESTATE5 -> SBR.STATE1 : [StatusSBR_5 == true]
    SBR.ESTATE3 -> SBR.ESTATE4 : [StatusSBR_3 == true]
    SBR.STATE1 -> SBR.ESTATE2 : [Control_50.C_55_PD_Sort == true && Sensors_50.O_50_Claw_Del == true && StatusSBR_1 == true]
  state Processing_RotationOnly
    state Config_ROnly
      entry:
      St_ROnly_1 = false;
      during:
      % FB6 Rotation Only - bloco ativo so neste modo
      if Control_100.C_105_Initialization && Control_100.C_105_Rotation
      St_ROnly_1 = true;
      else
      St_ROnly_1 = false;
      end
    state Aguarda_ROnly
      entry:
      St_ROnly_2 = false;
      during:
      % N1: condicoes para iniciar a rotacao
      if Sensors_100.O_100_PInit_Pos && Sensors_90.O_90_Claw_High && ~Actuators_100.F_102_RT_On
      St_ROnly_2 = true;
      else
      St_ROnly_2 = false;
      end
    state Girando_ROnly
      entry:
      St_ROnly_3 = false;
      during:
      % N2: mesa girando (contador C10, preset 6)
      if Actuators_100.F_102_RT_On
      St_ROnly_3 = true;
      else
      St_ROnly_3 = false;
      end
    state Retirada_ROnly
      entry:
      St_ROnly_5 = false;
      during:
      % N5: peca retirada pela garra da HD2, reseta o ciclo
      if Sensors_90.O_90_Claw_Del && Sensors_90.O_90_Claw_Low && Sensors_90.O_90_Part_in_Claw
      St_ROnly_5 = true;
      else
      St_ROnly_5 = false;
      end
    state RotacaoOK_ROnly
      entry:
      St_ROnly_4 = false;
      during:
      % N3/N4: fim da rotacao, peca pronta para retirada
      if ~Actuators_100.F_102_RT_On && Sensors_100.O_100_PInit_Pos
      St_ROnly_4 = true;
      else
      St_ROnly_4 = false;
      end
    Config_ROnly -> Aguarda_ROnly : [St_ROnly_1 == true]
    Aguarda_ROnly -> Girando_ROnly : [St_ROnly_2 == true]
    (default) -> Config_ROnly
    Girando_ROnly -> RotacaoOK_ROnly : [St_ROnly_3 == true]
    RotacaoOK_ROnly -> Retirada_ROnly : [St_ROnly_4 == true]
  note: Vision
  state Vision
    state FinishesProcess
      entry:
      St_Visn_5_13 = false;
      during:
      Control_90.C_95_PD_Proc;
      if Control_90.C_95_PD_Proc
      St_Visn_5_13 = true;
      else
      St_Visn_5_13 = false;
      end
    state InitialCondition
      entry:
      St_Visn_5_1 = false;
      during:
      AS_i_90.A_94_Cart_Full;
      Control_90.C_95_Initialization;
      Control_90.C_95_Cart2Del;
      Control_90.C_92_Profibus;
      Sensors_90.O_91_Key_Pos;
      if AS_i_90.A_94_Cart_Full && ...
      Control_90.C_95_Initialization && ...
      Control_90.C_95_Cart2Del && ...
      Control_90.C_92_Profibus && ...
      Sensors_90.O_91_Key_Pos
      St_Visn_5_1 = true;
      else
      St_Visn_5_1 = false;
      end
    (default) -> Vision.InitialCondition
    Vision.InitialCondition -> ? : [AS_i_90.A_94_CRoute_In == true && ...
        |  St_Visn_5_1 == true]
  note: Robot [30]
  state Robot1
    state InitialCondition
      entry:
      St_Rbt1_5_1 = false;
      during:
      AS_i_90.A_94_Cart_Full;
      Control_90.C_95_Initialization;
      Control_90.C_95_Cart2Del;
      Control_90.C_92_Profibus;
      Sensors_90.O_91_Key_Pos;
      if AS_i_90.A_94_Cart_Full && ...
      Control_90.C_95_Initialization && ...
      Control_90.C_95_Cart2Del && ...
      Control_90.C_92_Profibus && ...
      Sensors_90.O_91_Key_Pos
      St_Rbt1_5_1 = true;
      else
      St_Rbt1_5_1 = false;
      end
    state FinishesProcess
      entry:
      St_Rbt1_5_13 = false;
      during:
      Control_90.C_95_PD_Proc;
      if Control_90.C_95_PD_Proc
      St_Rbt1_5_13 = true;
      else
      St_Rbt1_5_13 = false;
      end
    (default) -> Robot1.InitialCondition
    Robot1.InitialCondition -> ? : [AS_i_90.A_94_CRoute_In == true && ...
        |  St_Rbt1_5_1 == true]
  note: Conveyor
  state CartToProcessing2
    state InitialCondition
      entry:
      St_C2P2_4_1 = false;
      during:
      Actuators_20.F_22_Conveyor;
      AS_i_70.A_74_Cart_Full;
      AS_i_70.A_73_TestCartID;
      AS_i_70.A_74_Pist_Bck;
      AS_i_70.A_74_Release_FB;
      if ~Actuators_20.F_22_Conveyor && ...
      AS_i_70.A_74_Cart_Full && ...
      ~AS_i_70.A_73_TestCartID ~= 0 && ...
      ~AS_i_70.A_74_Pist_Bck && ...
      ~AS_i_70.A_74_Release_FB
      St_C2P2_4_1 = true;
      else
      St_C2P2_4_1 = false;
      end
    state StartsProcess
      entry:
      St_C2P2_4_2 = false;
      during:
      Actuators_20.F_22_Conveyor;
      AS_i_70.A_73_TestCartID;
      AS_i_70.A_74_Pist_Bck;
      AS_i_70.A_74_Release_FB;
      if Actuators_20.F_22_Conveyor && ...
      AS_i_70.A_73_TestCartID == 0 && ...
      AS_i_70.A_74_Pist_Bck && ...
      AS_i_70.A_74_Release_FB
      St_C2P2_4_2 = true;
      else
      St_C2P2_4_2 = false;
      end
    state PartLeavesSensor
      entry:
      St_C2P2_4_3 = false;
      during:
      Actuators_70.F_73_Led_Extra2;
      AS_i_70.A_74_Cart_Full;
      AS_i_70.A_74_Optic;
      if ~Actuators_70.F_73_Led_Extra2 && ...
      ~AS_i_70.A_74_Cart_Full && ...
      ~AS_i_70.A_74_Optic
      St_C2P2_4_3 = true;
      else
      St_C2P2_4_3 = false;
      end
    state CartStartsMoving
      entry:
      St_C2P2_4_4 = false;
      during:
      Actuators_70.F_73_Led_Extra1;
      AS_i_70.A_74_No_Cart;
      AS_i_70.A_74_Cart_Stat;
      if Actuators_70.F_73_Led_Extra1 && ...
      AS_i_70.A_74_No_Cart && ...
      ~AS_i_70.A_74_Cart_Stat
      St_C2P2_4_4 = true;
      else
      St_C2P2_4_4 = false;
      end
    state CartGetsNearNextStation
      entry:
      St_C2P2_4_5 = false;
      during:
      AS_i_70.A_74_Cart_Next;
      AS_i_70.A_74_Pist_Bck;
      AS_i_70.A_74_Release_FB;
      if AS_i_70.A_74_Cart_Next && ...
      ~AS_i_70.A_74_Pist_Bck && ...
      ~AS_i_70.A_74_Release_FB
      St_C2P2_4_5 = true;
      else
      St_C2P2_4_5 = false;
      end
    state DetectionofCartNumberinStation
      entry:
      St_C2P2_4_6 = false;
      during:
      AS_i_90.A_93_ProcCartID
      if ~AS_i_90.A_93_ProcCartID ~=0
      St_C2P2_4_6 = true;
      else
      St_C2P2_4_6 = false;
      end
    state CartPassesNextStation
      entry:
      St_C2P2_4_7 = false;
      during:
      AS_i_70.A_74_Cart_Next
      if ~AS_i_70.A_74_Cart_Next
      St_C2P2_4_7 = true;
      else
      St_C2P2_4_7 = false;
      end
    state PartArrivesSensor
      entry:
      St_C2P2_4_8 = false;
      during:
      AS_i_90.A_94_Optic;
      if AS_i_90.A_94_Optic
      St_C2P2_4_8 = true;
      else
      St_C2P2_4_8 = false;
      end
    state CartArrivesinNextStation
      entry:
      St_C2P2_4_9 = false;
      during:
      Control_20.C_25_CartDel;
      Actuators_90.F_93_Led_Extra1;
      AS_i_90.A_94_Cart_Stat;
      AS_i_90.A_94_No_Cart;
      AS_i_90.A_94_Cart_Full;
      AS_i_90.A_94_CRoute_In;
      if Control_20.C_25_CartDel && ...
      ~Actuators_90.F_93_Led_Extra1 && ...
      AS_i_90.A_94_Cart_Stat && ...
      ~AS_i_90.A_94_No_Cart && ...
      AS_i_90.A_94_Cart_Full && ...
      AS_i_90.A_94_CRoute_In
      St_C2P2_4_9 = true;
      else
      St_C2P2_4_9 = false;
      end
    state T1
      during:
      Control_20.C_25_Request
    state T3
      during:
      Control_20.C_25_CartDel
    state T2
      during:
      AS_i_90.A_94_CRoute_In
    (default) -> CartToProcessing2.InitialCondition
    CartToProcessing2.DetectionofCartNumberinStation -> CartToProcessing2.CartPassesNextStation : [Sensors_20.O_24_Cart_Next == false && ...
        | St_C2P2_4_6 == true]
    CartToProcessing2.InitialCondition -> CartToProcessing2.StartsProcess : [Control_20.C_25_Request == true && ...
        |  St_C2P2_4_1 == true]
    CartToProcessing2.StartsProcess -> CartToProcessing2.PartLeavesSensor [order 1] : [Sensors_20.O_24_Optic == false && ...
        | St_C2P2_4_2 == true]
    CartToProcessing2.PartLeavesSensor -> CartToProcessing2.CartStartsMoving : [Sensors_20.O_24_Cart_Stat == false && ...
        | St_C2P2_4_3 == true]
    CartToProcessing2.CartStartsMoving -> CartToProcessing2.CartGetsNearNextStation : [Sensors_20.O_24_Cart_Next == true && ...
        | St_C2P2_4_4 == true]
    CartToProcessing2.CartGetsNearNextStation -> CartToProcessing2.DetectionofCartNumberinStation : [Sensors_20.O_24_Count == true && ...
        | St_C2P2_4_5 == true]
    CartToProcessing2.CartPassesNextStation -> CartToProcessing2.PartArrivesSensor : [Sensors_20.O_25_Optic == true && ...
        | St_C2P2_4_7 == true]
    CartToProcessing2.PartArrivesSensor -> CartToProcessing2.CartArrivesinNextStation : [Sensors_20.O_25_Cart_Stat == true && ...
        | St_C2P2_4_8 == true]
    CartToProcessing2.StartsProcess -> CartToProcessing2.T1 [order 2] : [after(2, sec)]
    CartToProcessing2.CartArrivesinNextStation -> (junction 1968)
    (junction 1968) -> CartToProcessing2.T3 [order 2] : [after(3,sec)]
    (junction 1968) -> CartToProcessing2.T2 [order 1] : [after(2,sec)]
  state Robot2
    state FinishesProcess
      entry:
      St_Rbt2_5_13 = false;
      during:
      Control_90.C_95_PD_Proc;
      if Control_90.C_95_PD_Proc
      St_Rbt2_5_13 = true;
      else
      St_Rbt2_5_13 = false;
      end
    state InitialCondition
      entry:
      St_Rbt2_5_1 = false;
      during:
      AS_i_90.A_94_Cart_Full;
      Control_90.C_95_Initialization;
      Control_90.C_95_Cart2Del;
      Control_90.C_92_Profibus;
      Sensors_90.O_91_Key_Pos;
      if AS_i_90.A_94_Cart_Full && ...
      Control_90.C_95_Initialization && ...
      Control_90.C_95_Cart2Del && ...
      Control_90.C_92_Profibus && ...
      Sensors_90.O_91_Key_Pos
      St_Rbt2_5_1 = true;
      else
      St_Rbt2_5_1 = false;
      end
    (default) -> Robot2.InitialCondition
    Robot2.InitialCondition -> ? : [AS_i_90.A_94_CRoute_In == true && ...
        |  St_Rbt2_5_1 == true]
  (default) -> Variable_Declaration [order 2]
  (default) -> Start [order 1]
  Start -> CartToTesting : [Control_20.C_24_Request == true]
  (junction 2436) -> BRS Output : [Control_60.C_65_BRS_Output == true]
  (junction 2433) -> (junction 2436) [order 2]
  (junction 2151) -> CartToTesting
  PartToProcessing2 -> (junction 2151) [order 2]
  CartToTesting -> (junction 1047) : [Control_20.C_24_CartDel == true]
  (junction 1047) -> (junction 1049)
  (junction 2433) -> BSR Output [order 1] : [Control_60.C_65_BSR_Output == true]
  (junction 2430) -> (junction 2433) [order 2]
  Distribution_Single -> (junction 829) : [Control_80.C_85_Part_Del == true]
  (junction 832) -> Identified_Delivery
  Identified_Delivery -> (junction 968) : [Control_70.C_75_Part_Del == true]
  (junction 829) -> (junction 826)
  (junction 831) -> (junction 832) [order 2] : [Control_70.C_75_Identified == true]
  (junction 968) -> (junction 971)
  (junction 729) -> (junction 999)
  (junction 999) -> Distribution_Single
  (junction 726) -> (junction 729) [order 1] : [Control_80.C_85_Single == true]
  (junction 993) -> (junction 999) : [Control_70.C_75_RQ_Wrong == true]
  (junction 2430) -> RBS Output [order 1] : [Control_60.C_65_RBS_Output == true]
  (junction 2420) -> (junction 2430) [order 1]
  (junction 971) -> (junction 1044)
  (junction 967) -> (junction 971)
  (junction 1044) -> CartToProcessing : [Control_20.C_25_Request == true]
  (junction 1049) -> (junction 726)
  (junction 726) -> (junction 996) [order 3] : [Control_80.C_85_Continuous == true]
  (junction 996) -> Distribution_Continuous
  Distribution_Continuous -> (junction 826) : [Control_80.C_85_Part_Del == true]
  (junction 826) -> (junction 831)
  (junction 726) -> (junction 732) [order 2] : [Control_80.C_85_Counted == true]
  (junction 992) -> (junction 996) [order 1] : [Control_70.C_75_RQ_Wrong == true]
  (junction 827) -> (junction 826)
  (junction 831) -> (junction 833) [order 1] : [Control_70.C_75_Requested == true]
  (junction 2143) -> PartToProcessing2
  CartToProcessing4 -> (junction 2143)
  PartToProcessing2 -> (junction 2420) [order 1] : [Control_50.C_55_PD_Sort == true]
  (junction 2420) -> (junction 2421) [order 2]
  (junction 2421) -> RSB Output [order 2] : [Control_60.C_65_RSB_Output == true]
  (junction 2421) -> (junction 2424) [order 1]
  Distribution_Counted -> (junction 827) : [Control_80.C_85_Part_Del == true]
  (junction 732) -> (junction 987)
  (junction 987) -> Distribution_Counted
  (junction 833) -> Requested_Delivery
  Requested_Delivery -> (junction 967) [order 1] : [Control_70.C_75_Part_Del == true]
  (junction 982) -> (junction 987) [order 1] : [Control_70.C_75_RQ_Wrong == true]
  PartToProcessing -> Processing_TestOnly [order 2] : [Control_90.C_95_PD_Proc == true && Control_100.C_105_Test == true]
  Processing_TestOnly -> PartToProcessing1 : [Control_100.C_105_Part_ready == true]
  Requested_Delivery -> (junction 965) [order 2] : [Control_70.C_75_RQ_Wrong == true]
  (junction 992) -> (junction 993) [order 2]
  (junction 982) -> (junction 992) [order 2]
  (junction 965) -> (junction 982)
  (junction 2424) -> SRB Output [order 2] : [Control_60.C_65_SRB_Output == true]
  (junction 2424) -> (junction 2427) [order 1]
  PartToProcessing -> Processing_TestDrill [order 3] : [Control_90.C_95_PD_Proc == true && Control_100.C_105_TestDrill == true]
  PartToProcessing -> Processing_RotationOnly [order 4] : [Control_90.C_95_PD_Proc == true && Control_100.C_105_Rotation == true]
  (junction 2141) -> CartToProcessing4
  (junction 2140) -> (junction 2141)
  (junction 2061) -> (junction 2140)
  (junction 2427) -> SBR Output : [Control_60.C_65_SBR_Output == true]
  Processing_TestDrill -> PartToProcessing1 : [Control_100.C_105_Part_ready == true]
  CartToProcessing -> (junction 1506) : [Control_20.C_25_CartDel == true]
  (junction 1830) -> ? [order 3]
  (junction 2064) -> Store Par
  Store Par -> (junction 2061)
  (junction 2060) -> (junction 2064) [order 1]
  (junction 2071) -> (junction 2061)
  (junction 1506) -> PartToProcessing
  PartToProcessing -> (junction 1830) [order 1]
  (junction 1830) -> (junction 1834) [order 1]
  Processing_RotationOnly -> PartToProcessing1 : [Control_100.C_105_Part_ready == true]
  (junction 2077) -> (junction 2060)
  CartToProcessing3 -> (junction 2077)
  (junction 2060) -> (junction 2074) [order 2]
  Retrieve Part -> (junction 2071)
  (junction 2074) -> Retrieve Part
  (junction 1858) -> PartToProcessing1
  (junction 1861) -> PartToProcessing1 [order 1]
  (junction 1861) -> CartToProcessing1 [order 2] : [Control_20.C_25_Request == true]
  (junction 2050) -> CartToProcessing3
  CartToProcessing1 -> (junction 2014) : [Control_20.C_25_CartDel == true]
  (junction 2048) -> (junction 2050)
  (junction 2045) -> (junction 2048)
  (default) -> ? [order 2] : [Sensors_90.O_90_Claw_High == true && ...
      | Status5_5 == true]
  (default) -> ? [order 1] : [Sensors_90.O_90_Claw_High == true && ...
      | Status5_12 == true]
  (default) -> ? [order 2] : [Sensors_90.O_90_Claw_Low && ...
      | Status5_11 == true]
  Vision -> (junction 2015)
  (junction 2015) -> (junction 2017)
  (junction 2014) -> Vision
  (junction 2037) -> Robot1
  Robot1 -> (junction 2045)
  (junction 2035) -> (junction 2037) [order 1]
  (junction 2043) -> (junction 2045)
  CartToProcessing2 -> (junction 2035)
  (junction 2035) -> (junction 2040) [order 2]
  (junction 2017) -> CartToProcessing2
  Robot2 -> (junction 2043)
  (junction 2040) -> Robot2
